simulink model "model"  (R2016a)
(part 10 of 11)

  _CN_91086220_220000_CN_24976300_220000/RConn3 -- T_24976300_380000;220000;110000_Umspannwerk_Pleinting/RConn3 -- Pleinting___Schwandorf_CN_24976300_220000_CN_28956649_220000/RConn3 -- L_24976300/LConn3
  _CN_91086220_220000_CN_77694901_220000/RConn1 -- T_77694901_220000;110000_Umspannwerk_Altheim/LConn1 -- Altheim___Sittling_CN_24759324_220000_CN_77694901_220000/LConn1
  _CN_91086220_220000_CN_77694901_220000/RConn2 -- T_77694901_220000;110000_Umspannwerk_Altheim/LConn2 -- Altheim___Sittling_CN_24759324_220000_CN_77694901_220000/LConn2
  _CN_91086220_220000_CN_77694901_220000/RConn3 -- T_77694901_220000;110000_Umspannwerk_Altheim/LConn3 -- Altheim___Sittling_CN_24759324_220000_CN_77694901_220000/LConn3
  _CN_152924498_220000_CN152506744/RConn1 -- G_152506744_Großkraftwerk_Mannheim/RConn1 -- _CN_163093653_220000_CN152506744/LConn1
  _CN_152924498_220000_CN152506744/RConn2 -- G_152506744_Großkraftwerk_Mannheim/RConn2 -- _CN_163093653_220000_CN152506744/LConn2
  _CN_152924498_220000_CN152506744/RConn3 -- G_152506744_Großkraftwerk_Mannheim/RConn3 -- _CN_163093653_220000_CN152506744/LConn3
  220kV_Fichtenhain_West+Utfort_West_CN_93278553_220000_CN_24815262_220000/LConn1 -- T_93278553_220000;110000_Station_Edelstahl_Krefeld/LConn1 -- 220kV_Fichtenhain_West+Utfort_West_CN_93278553_220000_CN_24799890_220000/RConn1 -- 220kV_Fichtenhain_West+Utfort_West_CN_93278553_220000_CN_23380800_220000/LConn1 -- 220kV_Fichtenhain_West+Utfort_West_CN_93278553_220000_CN92877616/LConn1 -- 220kV_Fichtenhain_West+Utfort_West_CN_93278553_220000_CN_91854336_220000/RConn1 -- 220kV_Fichtenhain_West+Utfort_West_CN_93278553_220000_CN_24479984_220000/LConn1
  220kV_Fichtenhain_West+Utfort_West_CN_93278553_220000_CN_24815262_220000/LConn2 -- T_93278553_220000;110000_Station_Edelstahl_Krefeld/LConn2 -- 220kV_Fichtenhain_West+Utfort_West_CN_93278553_220000_CN_24799890_220000/RConn2 -- 220kV_Fichtenhain_West+Utfort_West_CN_93278553_220000_CN_23380800_220000/LConn2 -- 220kV_Fichtenhain_West+Utfort_West_CN_93278553_220000_CN92877616/LConn2 -- 220kV_Fichtenhain_West+Utfort_West_CN_93278553_220000_CN_91854336_220000/RConn2 -- 220kV_Fichtenhain_West+Utfort_West_CN_93278553_220000_CN_24479984_220000/LConn2
  220kV_Fichtenhain_West+Utfort_West_CN_93278553_220000_CN_24815262_220000/LConn3 -- T_93278553_220000;110000_Station_Edelstahl_Krefeld/LConn3 -- 220kV_Fichtenhain_West+Utfort_West_CN_93278553_220000_CN_24799890_220000/RConn3 -- 220kV_Fichtenhain_West+Utfort_West_CN_93278553_220000_CN_23380800_220000/LConn3 -- 220kV_Fichtenhain_West+Utfort_West_CN_93278553_220000_CN92877616/LConn3 -- 220kV_Fichtenhain_West+Utfort_West_CN_93278553_220000_CN_91854336_220000/RConn3 -- 220kV_Fichtenhain_West+Utfort_West_CN_93278553_220000_CN_24479984_220000/LConn3
  220kV_Fichtenhain_West+Utfort_West_CN_93278553_220000_CN_24815262_220000/RConn1 -- T_24815262_380000;220000;110000_Station_Dülken/RConn1 -- L_24815262/LConn1
  220kV_Fichtenhain_West+Utfort_West_CN_93278553_220000_CN_24815262_220000/RConn2 -- T_24815262_380000;220000;110000_Station_Dülken/RConn2 -- L_24815262/LConn2
  220kV_Fichtenhain_West+Utfort_West_CN_93278553_220000_CN_24815262_220000/RConn3 -- T_24815262_380000;220000;110000_Station_Dülken/RConn3 -- L_24815262/LConn3
  220kV_Fichtenhain_West+Utfort_West_CN_93278553_220000_CN_23380800_220000/RConn1 -- T_23380800_380000;220000;110000_Station_Utfort/RConn1 -- 220kV_Wesel_Ost_CN_24462426_220000_CN_23380800_220000/RConn1 -- L_23380800/LConn1
  220kV_Fichtenhain_West+Utfort_West_CN_93278553_220000_CN_23380800_220000/RConn2 -- T_23380800_380000;220000;110000_Station_Utfort/RConn2 -- 220kV_Wesel_Ost_CN_24462426_220000_CN_23380800_220000/RConn2 -- L_23380800/LConn2
  220kV_Fichtenhain_West+Utfort_West_CN_93278553_220000_CN_23380800_220000/RConn3 -- T_23380800_380000;220000;110000_Station_Utfort/RConn3 -- 220kV_Wesel_Ost_CN_24462426_220000_CN_23380800_220000/RConn3 -- L_23380800/LConn3
  G_92877616_Kraftwerk_Huckingen/RConn1 -- 220kV_Fichtenhain_West+Utfort_West_CN_93278553_220000_CN92877616/RConn1
  G_92877616_Kraftwerk_Huckingen/RConn2 -- 220kV_Fichtenhain_West+Utfort_West_CN_93278553_220000_CN92877616/RConn2
  G_92877616_Kraftwerk_Huckingen/RConn3 -- 220kV_Fichtenhain_West+Utfort_West_CN_93278553_220000_CN92877616/RConn3
  T_24479984_220000;110000_Uerdingen/LConn1 -- 220kV_Fichtenhain_West+Utfort_West_CN_93278553_220000_CN_24479984_220000/RConn1
  T_24479984_220000;110000_Uerdingen/LConn2 -- 220kV_Fichtenhain_West+Utfort_West_CN_93278553_220000_CN_24479984_220000/RConn2
  T_24479984_220000;110000_Uerdingen/LConn3 -- 220kV_Fichtenhain_West+Utfort_West_CN_93278553_220000_CN_24479984_220000/RConn3
  T_74893659_380000;110000_HGÜ_Baltic_Cable___Stromrichterstation_Herrenwyk/LConn1 -- _CN_74893659_380000_CN_74893662_380000/LConn1
  T_74893659_380000;110000_HGÜ_Baltic_Cable___Stromrichterstation_Herrenwyk/LConn2 -- _CN_74893659_380000_CN_74893662_380000/LConn2
  T_74893659_380000;110000_HGÜ_Baltic_Cable___Stromrichterstation_Herrenwyk/LConn3 -- _CN_74893659_380000_CN_74893662_380000/LConn3
  T_74893662_380000;220000;110000_Umspannwerk_Siems/LConn1 -- _CN_74893659_380000_CN_74893662_380000/RConn1
  T_74893662_380000;220000;110000_Umspannwerk_Siems/LConn2 -- _CN_74893659_380000_CN_74893662_380000/RConn2
  T_74893662_380000;220000;110000_Umspannwerk_Siems/LConn3 -- _CN_74893659_380000_CN_74893662_380000/RConn3
  Scholven_C_CN_38584673_220000_CN22943608/RConn1 -- G_22943608_Kraftwerk_Scholven/RConn1 -- 220kV_Scholven_E_CN_23022100_220000_CN22943608/RConn1 -- 380kV_Scholven_B_CN_23022100_380000_CN22943608/RConn1
  Scholven_C_CN_38584673_220000_CN22943608/RConn2 -- G_22943608_Kraftwerk_Scholven/RConn2 -- 220kV_Scholven_E_CN_23022100_220000_CN22943608/RConn2 -- 380kV_Scholven_B_CN_23022100_380000_CN22943608/RConn2
  Scholven_C_CN_38584673_220000_CN22943608/RConn3 -- G_22943608_Kraftwerk_Scholven/RConn3 -- 220kV_Scholven_E_CN_23022100_220000_CN22943608/RConn3 -- 380kV_Scholven_B_CN_23022100_380000_CN22943608/RConn3
  T_89352550_380000;220000;110000_Bexbach_Kraftwerk/LConn1 -- _CN_89352550_380000_CN28051874/RConn1
  T_89352550_380000;220000;110000_Bexbach_Kraftwerk/LConn2 -- _CN_89352550_380000_CN28051874/RConn2
  T_89352550_380000;220000;110000_Bexbach_Kraftwerk/LConn3 -- _CN_89352550_380000_CN28051874/RConn3
  _CN_89352550_220000_CN28051874/RConn1 -- T_89352550_380000;220000;110000_Bexbach_Kraftwerk/RConn1 -- L_89352550/LConn1
  _CN_89352550_220000_CN28051874/RConn2 -- T_89352550_380000;220000;110000_Bexbach_Kraftwerk/RConn2 -- L_89352550/LConn2
  _CN_89352550_220000_CN28051874/RConn3 -- T_89352550_380000;220000;110000_Bexbach_Kraftwerk/RConn3 -- L_89352550/LConn3
  220_kV_Bigge_Ost|West_CN_22761839_220000_CN_24667346_220000/RConn1 -- T_24667346_220000;110000_Umspannwerk_Garenfeld/LConn1 -- _CN_66038431_220000_CN_24667346_220000/LConn1 -- 220kV_Nordleitung_CN_24667346_220000_CN_83916207_220000/LConn1
  220_kV_Bigge_Ost|West_CN_22761839_220000_CN_24667346_220000/RConn2 -- T_24667346_220000;110000_Umspannwerk_Garenfeld/LConn2 -- _CN_66038431_220000_CN_24667346_220000/LConn2 -- 220kV_Nordleitung_CN_24667346_220000_CN_83916207_220000/LConn2
  220_kV_Bigge_Ost|West_CN_22761839_220000_CN_24667346_220000/RConn3 -- T_24667346_220000;110000_Umspannwerk_Garenfeld/LConn3 -- _CN_66038431_220000_CN_24667346_220000/LConn3 -- 220kV_Nordleitung_CN_24667346_220000_CN_83916207_220000/LConn3
  T_51940126_220000;110000_Umspannwerk_Bixterheide/LConn1 -- 220_kV_Bigge_Ost|West_CN_22761839_220000_CN_51940126_220000/RConn1
  T_51940126_220000;110000_Umspannwerk_Bixterheide/LConn2 -- 220_kV_Bigge_Ost|West_CN_22761839_220000_CN_51940126_220000/RConn2
  T_51940126_220000;110000_Umspannwerk_Bixterheide/LConn3 -- 220_kV_Bigge_Ost|West_CN_22761839_220000_CN_51940126_220000/RConn3
  220_kV_Bigge_Ost|West_CN_22761839_220000_CN_132814303_220000/RConn1 -- T_132814303_220000;110000_Station_Altenkleusheim/LConn1 -- 220kV_Siegerland_West_CN_89043564_220000_CN_132814303_220000/LConn1
  220_kV_Bigge_Ost|West_CN_22761839_220000_CN_132814303_220000/RConn2 -- T_132814303_220000;110000_Station_Altenkleusheim/LConn2 -- 220kV_Siegerland_West_CN_89043564_220000_CN_132814303_220000/LConn2
  220_kV_Bigge_Ost|West_CN_22761839_220000_CN_132814303_220000/RConn3 -- T_132814303_220000;110000_Station_Altenkleusheim/LConn3 -- 220kV_Siegerland_West_CN_89043564_220000_CN_132814303_220000/LConn3
  T_22761692_220000;110000_UW_Fühlingen/LConn1 -- 220_kV_Niederaußem_4d;_Wiesdorf_Ltg__CN_22761839_220000_CN_22761692_220000/RConn1
  T_22761692_220000;110000_UW_Fühlingen/LConn2 -- 220_kV_Niederaußem_4d;_Wiesdorf_Ltg__CN_22761839_220000_CN_22761692_220000/RConn2
  T_22761692_220000;110000_UW_Fühlingen/LConn3 -- 220_kV_Niederaußem_4d;_Wiesdorf_Ltg__CN_22761839_220000_CN_22761692_220000/RConn3
  220_kV_Niederaußem_4d;_Wiesdorf_Ltg__CN_22761839_220000_CN_24839976_220000/RConn1 -- T_24839976_380000;220000_Umspannwerk_Rommerskirchen/RConn1 -- 220_kV_Rommerskirchen_Ost_CN_24839976_220000_CN_23084554_220000/LConn1 -- 220_kV_Frixheim_Nord|Süd_CN_24839976_220000_CN_27919734_220000/LConn1 -- L_24839976/LConn1
  220_kV_Niederaußem_4d;_Wiesdorf_Ltg__CN_22761839_220000_CN_24839976_220000/RConn2 -- T_24839976_380000;220000_Umspannwerk_Rommerskirchen/RConn2 -- 220_kV_Rommerskirchen_Ost_CN_24839976_220000_CN_23084554_220000/LConn2 -- 220_kV_Frixheim_Nord|Süd_CN_24839976_220000_CN_27919734_220000/LConn2 -- L_24839976/LConn2
  220_kV_Niederaußem_4d;_Wiesdorf_Ltg__CN_22761839_220000_CN_24839976_220000/RConn3 -- T_24839976_380000;220000_Umspannwerk_Rommerskirchen/RConn3 -- 220_kV_Rommerskirchen_Ost_CN_24839976_220000_CN_23084554_220000/LConn3 -- 220_kV_Frixheim_Nord|Süd_CN_24839976_220000_CN_27919734_220000/LConn3 -- L_24839976/LConn3
  220_kV_Niederaußem_4d;_Wiesdorf_Ltg__CN_22761839_220000_CN24840439/RConn1 -- G_24840439_Kraftwerk_Niederaussem/RConn1 -- 220_kV_Niederaußem_3c_CN_32993727_220000_CN24840439/LConn1 -- _CN_24839976_380000_CN24840439/RConn1
  220_kV_Niederaußem_4d;_Wiesdorf_Ltg__CN_22761839_220000_CN24840439/RConn2 -- G_24840439_Kraftwerk_Niederaussem/RConn2 -- 220_kV_Niederaußem_3c_CN_32993727_220000_CN24840439/LConn2 -- _CN_24839976_380000_CN24840439/RConn2
  220_kV_Niederaußem_4d;_Wiesdorf_Ltg__CN_22761839_220000_CN24840439/RConn3 -- G_24840439_Kraftwerk_Niederaussem/RConn3 -- 220_kV_Niederaußem_3c_CN_32993727_220000_CN24840439/LConn3 -- _CN_24839976_380000_CN24840439/RConn3
  T_22764922_220000;110000_Station_Dhünnaue/LConn1 -- 220_kV_Niederaußem_4d;_Wiesdorf_Ltg__CN_22761839_220000_CN_22764922_220000/RConn1
  T_22764922_220000;110000_Station_Dhünnaue/LConn2 -- 220_kV_Niederaußem_4d;_Wiesdorf_Ltg__CN_22761839_220000_CN_22764922_220000/RConn2
  T_22764922_220000;110000_Station_Dhünnaue/LConn3 -- 220_kV_Niederaußem_4d;_Wiesdorf_Ltg__CN_22761839_220000_CN_22764922_220000/RConn3
  380_kV_Neurath_2b;_Oerkhaus_Ost_CN_22761839_380000_CN_49577448_380000/RConn1 -- T_49577448_380000;220000_Station_Sankt_Peter_380_kV/LConn1 -- 380kV_Knechtsteden_West_CN_77179271_380000_CN_49577448_380000/LConn1
  380_kV_Neurath_2b;_Oerkhaus_Ost_CN_22761839_380000_CN_49577448_380000/RConn2 -- T_49577448_380000;220000_Station_Sankt_Peter_380_kV/LConn2 -- 380kV_Knechtsteden_West_CN_77179271_380000_CN_49577448_380000/LConn2
  380_kV_Neurath_2b;_Oerkhaus_Ost_CN_22761839_380000_CN_49577448_380000/RConn3 -- T_49577448_380000;220000_Station_Sankt_Peter_380_kV/LConn3 -- 380kV_Knechtsteden_West_CN_77179271_380000_CN_49577448_380000/LConn3
  T_106096507_380000;110000_Station_Ohligs/LConn1 -- 380_kV_Neurath_2b;_Oerkhaus_Ost_CN_22761839_380000_CN_106096507_380000/RConn1
  T_106096507_380000;110000_Station_Ohligs/LConn2 -- 380_kV_Neurath_2b;_Oerkhaus_Ost_CN_22761839_380000_CN_106096507_380000/RConn2
  T_106096507_380000;110000_Station_Ohligs/LConn3 -- 380_kV_Neurath_2b;_Oerkhaus_Ost_CN_22761839_380000_CN_106096507_380000/RConn3
  380kV_Sauerland_Süd_CN_42799487_380000_CN_42488850_380000/RConn1 -- T_42799487_380000;110000_Station_Arpe/LConn1 -- 380kV_Sauerland_Süd_CN_42799487_380000_CN_42797575_380000/LConn1
  380kV_Sauerland_Süd_CN_42799487_380000_CN_42488850_380000/RConn2 -- T_42799487_380000;110000_Station_Arpe/LConn2 -- 380kV_Sauerland_Süd_CN_42799487_380000_CN_42797575_380000/LConn2
  380kV_Sauerland_Süd_CN_42799487_380000_CN_42488850_380000/RConn3 -- T_42799487_380000;110000_Station_Arpe/LConn3 -- 380kV_Sauerland_Süd_CN_42799487_380000_CN_42797575_380000/LConn3
  380kV_Sauerland_Süd_CN_42799487_380000_CN_42797575_380000/RConn1 -- T_42797575_380000;110000_Station_Nehden/LConn1 -- 380kV_Twistetal_Ost_3_CN_42797575_380000_CN_41232144_380000/LConn1 -- 380kV_Twistetal_Ost_3_CN_42797575_380000_CN_25943440_380000/LConn1
  380kV_Sauerland_Süd_CN_42799487_380000_CN_42797575_380000/RConn2 -- T_42797575_380000;110000_Station_Nehden/LConn2 -- 380kV_Twistetal_Ost_3_CN_42797575_380000_CN_41232144_380000/LConn2 -- 380kV_Twistetal_Ost_3_CN_42797575_380000_CN_25943440_380000/LConn2
  380kV_Sauerland_Süd_CN_42799487_380000_CN_42797575_380000/RConn3 -- T_42797575_380000;110000_Station_Nehden/LConn3 -- 380kV_Twistetal_Ost_3_CN_42797575_380000_CN_41232144_380000/LConn3 -- 380kV_Twistetal_Ost_3_CN_42797575_380000_CN_25943440_380000/LConn3
  380kV_Knechtsteden_West_CN_77179271_380000_CN_24839976_380000/RConn1 -- T_77179271_380000_Station_Osterath/LConn1 -- 380kV_Meerbusch_West_CN_77179271_380000_CN_25044557_380000/LConn1 -- 380kV_Knechtsteden_West_CN_77179271_380000_CN_49577448_380000/RConn1 -- 380kV_Knechtsteden_West_CN_77179271_380000_CN_95434457_380000/LConn1 -- 380kV_Knechtsteden_West_CN_77179271_380000_CN109373271/LConn1 -- 380kV_Meerbusch_West_CN_77179271_380000_CN_23380800_380000/LConn1
  380kV_Knechtsteden_West_CN_77179271_380000_CN_24839976_380000/RConn2 -- T_77179271_380000_Station_Osterath/LConn2 -- 380kV_Meerbusch_West_CN_77179271_380000_CN_25044557_380000/LConn2 -- 380kV_Knechtsteden_West_CN_77179271_380000_CN_49577448_380000/RConn2 -- 380kV_Knechtsteden_West_CN_77179271_380000_CN_95434457_380000/LConn2 -- 380kV_Knechtsteden_West_CN_77179271_380000_CN109373271/LConn2 -- 380kV_Meerbusch_West_CN_77179271_380000_CN_23380800_380000/LConn2
  380kV_Knechtsteden_West_CN_77179271_380000_CN_24839976_380000/RConn3 -- T_77179271_380000_Station_Osterath/LConn3 -- 380kV_Meerbusch_West_CN_77179271_380000_CN_25044557_380000/LConn3 -- 380kV_Knechtsteden_West_CN_77179271_380000_CN_49577448_380000/RConn3 -- 380kV_Knechtsteden_West_CN_77179271_380000_CN_95434457_380000/LConn3 -- 380kV_Knechtsteden_West_CN_77179271_380000_CN109373271/LConn3 -- 380kV_Meerbusch_West_CN_77179271_380000_CN_23380800_380000/LConn3
  T_95434457_380000;220000;110000_KW_Neurath/LConn1 -- 380kV_Knechtsteden_West_CN_77179271_380000_CN_95434457_380000/RConn1
  T_95434457_380000;220000;110000_KW_Neurath/LConn2 -- 380kV_Knechtsteden_West_CN_77179271_380000_CN_95434457_380000/RConn2
  T_95434457_380000;220000;110000_KW_Neurath/LConn3 -- 380kV_Knechtsteden_West_CN_77179271_380000_CN_95434457_380000/RConn3
  G_109373271_RWE_Kraftwerk_Neurath_BoA_Bl__F_G/RConn1 -- 380kV_Knechtsteden_West_CN_77179271_380000_CN109373271/RConn1
  G_109373271_RWE_Kraftwerk_Neurath_BoA_Bl__F_G/RConn2 -- 380kV_Knechtsteden_West_CN_77179271_380000_CN109373271/RConn2
  G_109373271_RWE_Kraftwerk_Neurath_BoA_Bl__F_G/RConn3 -- 380kV_Knechtsteden_West_CN_77179271_380000_CN109373271/RConn3
  380kV_Meerbusch_West_CN_77179271_380000_CN_23380800_380000/RConn1 -- T_23380800_380000;220000;110000_Station_Utfort/LConn1 -- 380kV_Lohheide_West_CN_23380800_380000_CN26623135/RConn1
  380kV_Meerbusch_West_CN_77179271_380000_CN_23380800_380000/RConn2 -- T_23380800_380000;220000;110000_Station_Utfort/LConn2 -- 380kV_Lohheide_West_CN_23380800_380000_CN26623135/RConn2
  380kV_Meerbusch_West_CN_77179271_380000_CN_23380800_380000/RConn3 -- T_23380800_380000;220000;110000_Station_Utfort/LConn3 -- 380kV_Lohheide_West_CN_23380800_380000_CN26623135/RConn3
  T_25044557_380000_Station_Rath/LConn1 -- 380kV_Meerbusch_West_CN_77179271_380000_CN_25044557_380000/RConn1
  T_25044557_380000_Station_Rath/LConn2 -- 380kV_Meerbusch_West_CN_77179271_380000_CN_25044557_380000/RConn2
  T_25044557_380000_Station_Rath/LConn3 -- 380kV_Meerbusch_West_CN_77179271_380000_CN_25044557_380000/RConn3
  G_178167136_Kraftwerk_Boxberg/RConn1 -- MP_CN_157806991_380000_CN178167136/RConn1
  G_178167136_Kraftwerk_Boxberg/RConn2 -- MP_CN_157806991_380000_CN178167136/RConn2
  G_178167136_Kraftwerk_Boxberg/RConn3 -- MP_CN_157806991_380000_CN178167136/RConn3
  557_CN_157806991_380000_CN_157328339_380000/RConn1 -- T_157328339_380000;110000_Umspannwerk_Streumen/LConn1 -- 585_CN_157328339_380000_CN_32843531_380000/RConn1 -- 559_CN_157328339_380000_CN_23025610_380000/RConn1 -- 572_CN_23117075_380000_CN_157328339_380000/RConn1 -- 561_Streumen_CN_156683994_380000_CN_157328339_380000/RConn1
  557_CN_157806991_380000_CN_157328339_380000/RConn2 -- T_157328339_380000;110000_Umspannwerk_Streumen/LConn2 -- 585_CN_157328339_380000_CN_32843531_380000/RConn2 -- 559_CN_157328339_380000_CN_23025610_380000/RConn2 -- 572_CN_23117075_380000_CN_157328339_380000/RConn2 -- 561_Streumen_CN_156683994_380000_CN_157328339_380000/RConn2
  557_CN_157806991_380000_CN_157328339_380000/RConn3 -- T_157328339_380000;110000_Umspannwerk_Streumen/LConn3 -- 585_CN_157328339_380000_CN_32843531_380000/RConn3 -- 559_CN_157328339_380000_CN_23025610_380000/RConn3 -- 572_CN_23117075_380000_CN_157328339_380000/RConn3 -- 561_Streumen_CN_156683994_380000_CN_157328339_380000/RConn3
  552_CN_157806991_380000_CN_157807291_380000/RConn1 -- T_157807291_380000;110000_Umspannwerk_Schmölln/LConn1 -- Schmölln___Dresden_Süd___Röhrsdorf_CN_157807291_380000_CN_109917397_380000/LConn1 -- Schmölln___Dresden_Süd___Röhrsdorf_CN_157807291_380000_CN_23117075_380000/RConn1 -- Schmölln___Dresden_Süd___Röhrsdorf_CN_157807291_380000_CN_23241863_380000/LConn1 -- _CN_59026005_380000_CN_157807291_380000/LConn1
  552_CN_157806991_380000_CN_157807291_380000/RConn2 -- T_157807291_380000;110000_Umspannwerk_Schmölln/LConn2 -- Schmölln___Dresden_Süd___Röhrsdorf_CN_157807291_380000_CN_109917397_380000/LConn2 -- Schmölln___Dresden_Süd___Röhrsdorf_CN_157807291_380000_CN_23117075_380000/RConn2 -- Schmölln___Dresden_Süd___Röhrsdorf_CN_157807291_380000_CN_23241863_380000/LConn2 -- _CN_59026005_380000_CN_157807291_380000/LConn2
  552_CN_157806991_380000_CN_157807291_380000/RConn3 -- T_157807291_380000;110000_Umspannwerk_Schmölln/LConn3 -- Schmölln___Dresden_Süd___Röhrsdorf_CN_157807291_380000_CN_109917397_380000/LConn3 -- Schmölln___Dresden_Süd___Röhrsdorf_CN_157807291_380000_CN_23117075_380000/RConn3 -- Schmölln___Dresden_Süd___Röhrsdorf_CN_157807291_380000_CN_23241863_380000/LConn3 -- _CN_59026005_380000_CN_157807291_380000/LConn3
  _CN_25557397_380000_CN_43688805_380000/RConn1 -- T_43688805_380000;220000;110000_380kV_Umspannwerk_Pulverdingen/LConn1 -- Philippsburg___Pulverdingen_CN_43688805_380000_CN_254326606_380000/LConn1 -- Philippsburg___Pulverdingen_CN_43688805_380000_CN161909939/RConn1 -- 380_kV_CN_26260052_380000_CN_43688805_380000/LConn1 -- 2x_380_kV_CN_43688805_380000_CN_26814283_380000/LConn1
  _CN_25557397_380000_CN_43688805_380000/RConn2 -- T_43688805_380000;220000;110000_380kV_Umspannwerk_Pulverdingen/LConn2 -- Philippsburg___Pulverdingen_CN_43688805_380000_CN_254326606_380000/LConn2 -- Philippsburg___Pulverdingen_CN_43688805_380000_CN161909939/RConn2 -- 380_kV_CN_26260052_380000_CN_43688805_380000/LConn2 -- 2x_380_kV_CN_43688805_380000_CN_26814283_380000/LConn2
  _CN_25557397_380000_CN_43688805_380000/RConn3 -- T_43688805_380000;220000;110000_380kV_Umspannwerk_Pulverdingen/LConn3 -- Philippsburg___Pulverdingen_CN_43688805_380000_CN_254326606_380000/LConn3 -- Philippsburg___Pulverdingen_CN_43688805_380000_CN161909939/RConn3 -- 380_kV_CN_26260052_380000_CN_43688805_380000/LConn3 -- 2x_380_kV_CN_43688805_380000_CN_26814283_380000/LConn3
  G_146723308_Kernkraftwerk_Obrigheim,_stillgelegt/RConn1 -- _CN_25557397_220000_CN146723308/RConn1
  G_146723308_Kernkraftwerk_Obrigheim,_stillgelegt/RConn2 -- _CN_25557397_220000_CN146723308/RConn2
  G_146723308_Kernkraftwerk_Obrigheim,_stillgelegt/RConn3 -- _CN_25557397_220000_CN146723308/RConn3
  _CN_25557397_220000_CN_42050342_220000/RConn1 -- T_42050342_380000;220000;110000_Umspannwerk_Goldshöfe/RConn1 -- L_42050342/LConn1
  _CN_25557397_220000_CN_42050342_220000/RConn2 -- T_42050342_380000;220000;110000_Umspannwerk_Goldshöfe/RConn2 -- L_42050342/LConn2
  _CN_25557397_220000_CN_42050342_220000/RConn3 -- T_42050342_380000;220000;110000_Umspannwerk_Goldshöfe/RConn3 -- L_42050342/LConn3
  _CN_25557397_380000_CN89183108/RConn1 -- G_89183108_Heizkraftwerk_Heilbronn/RConn1 -- _CN_25557397_220000_CN89183108/RConn1
  _CN_25557397_380000_CN89183108/RConn2 -- G_89183108_Heizkraftwerk_Heilbronn/RConn2 -- _CN_25557397_220000_CN89183108/RConn2
  _CN_25557397_380000_CN89183108/RConn3 -- G_89183108_Heizkraftwerk_Heilbronn/RConn3 -- _CN_25557397_220000_CN89183108/RConn3
  T_104878489_220000;110000_Umspannwerk_Kraftwerk_Emden/LConn1 -- _CN_104878489_220000_CN_34835258_220000/LConn1
  T_104878489_220000;110000_Umspannwerk_Kraftwerk_Emden/LConn2 -- _CN_104878489_220000_CN_34835258_220000/LConn2
  T_104878489_220000;110000_Umspannwerk_Kraftwerk_Emden/LConn3 -- _CN_104878489_220000_CN_34835258_220000/LConn3
  _CN_104878489_220000_CN_34835258_220000/RConn1 -- T_34835258_220000;110000_Emden_Borßum/LConn1 -- 203_CN_34835258_220000_CN_173178563_220000/LConn1
  _CN_104878489_220000_CN_34835258_220000/RConn2 -- T_34835258_220000;110000_Emden_Borßum/LConn2 -- 203_CN_34835258_220000_CN_173178563_220000/LConn2
  _CN_104878489_220000_CN_34835258_220000/RConn3 -- T_34835258_220000;110000_Emden_Borßum/LConn3 -- 203_CN_34835258_220000_CN_173178563_220000/LConn3
  Wolkramshausen_CN_143882655_220000_CN_157164284_220000/LConn1 -- T_143882655_380000;220000;110000_Umspannwerk_Vieselbach/RConn1 -- L_143882655/LConn1
  Wolkramshausen_CN_143882655_220000_CN_157164284_220000/LConn2 -- T_143882655_380000;220000;110000_Umspannwerk_Vieselbach/RConn2 -- L_143882655/LConn2
  Wolkramshausen_CN_143882655_220000_CN_157164284_220000/LConn3 -- T_143882655_380000;220000;110000_Umspannwerk_Vieselbach/RConn3 -- L_143882655/LConn3
  Wolkramshausen_CN_143882655_220000_CN_157164284_220000/RConn1 -- T_157164284_220000_Wolkramshausen_(220_kV)/LConn1 -- 358_CN_157164284_220000_CN_22879599_220000/LConn1
  Wolkramshausen_CN_143882655_220000_CN_157164284_220000/RConn2 -- T_157164284_220000_Wolkramshausen_(220_kV)/LConn2 -- 358_CN_157164284_220000_CN_22879599_220000/LConn2
  Wolkramshausen_CN_143882655_220000_CN_157164284_220000/RConn3 -- T_157164284_220000_Wolkramshausen_(220_kV)/LConn3 -- 358_CN_157164284_220000_CN_22879599_220000/LConn3
  _CN_143882655_380000_CN_29309786_380000/RConn1 -- T_29309786_380000;110000_Mecklar/LConn1 -- _CN_29309786_380000_CN_156673636_380000/LConn1 -- _CN_29309786_380000_CN_148446247_380000/LConn1
  _CN_143882655_380000_CN_29309786_380000/RConn2 -- T_29309786_380000;110000_Mecklar/LConn2 -- _CN_29309786_380000_CN_156673636_380000/LConn2 -- _CN_29309786_380000_CN_148446247_380000/LConn2
  _CN_143882655_380000_CN_29309786_380000/RConn3 -- T_29309786_380000;110000_Mecklar/LConn3 -- _CN_29309786_380000_CN_156673636_380000/LConn3 -- _CN_29309786_380000_CN_148446247_380000/LConn3
  T_154418450_380000;110000_Eisenach/LConn1 -- _CN_143882655_380000_CN_154418450_380000/RConn1
  T_154418450_380000;110000_Eisenach/LConn2 -- _CN_143882655_380000_CN_154418450_380000/RConn2
  T_154418450_380000;110000_Eisenach/LConn3 -- _CN_143882655_380000_CN_154418450_380000/RConn3
  T_148211527_380000;110000_Großschwabhausen/LConn1 -- _CN_143882655_380000_CN_148211527_380000/RConn1
  T_148211527_380000;110000_Großschwabhausen/LConn2 -- _CN_143882655_380000_CN_148211527_380000/RConn2
  T_148211527_380000;110000_Großschwabhausen/LConn3 -- _CN_143882655_380000_CN_148211527_380000/RConn3
  T_24267175_220000;110000_Umspannanlage_Frimmersdorf_I/LConn1 -- _CN_24267175_220000_CN24267119/LConn1
  T_24267175_220000;110000_Umspannanlage_Frimmersdorf_I/LConn2 -- _CN_24267175_220000_CN24267119/LConn2
  T_24267175_220000;110000_Umspannanlage_Frimmersdorf_I/LConn3 -- _CN_24267175_220000_CN24267119/LConn3
  _CN_24267175_220000_CN24267119/RConn1 -- G_24267119_RWE_Kraftwerk_Frimmersdorf/RConn1 -- 220_kV_Neurath_1a_CN_27919734_220000_CN24267119/LConn1
  _CN_24267175_220000_CN24267119/RConn2 -- G_24267119_RWE_Kraftwerk_Frimmersdorf/RConn2 -- 220_kV_Neurath_1a_CN_27919734_220000_CN24267119/LConn2
  _CN_24267175_220000_CN24267119/RConn3 -- G_24267119_RWE_Kraftwerk_Frimmersdorf/RConn3 -- 220_kV_Neurath_1a_CN_27919734_220000_CN24267119/LConn3
  T_151507370_220000_/LConn1 -- _CN_151507370_220000_CN_28227099_220000/RConn1
  T_151507370_220000_/LConn2 -- _CN_151507370_220000_CN_28227099_220000/RConn2
  T_151507370_220000_/LConn3 -- _CN_151507370_220000_CN_28227099_220000/RConn3
  T_266684854_380000_Umspannwerk_Farge/LConn1 -- _CN_266684854_380000_CN313937042/RConn1
  T_266684854_380000_Umspannwerk_Farge/LConn2 -- _CN_266684854_380000_CN313937042/RConn2
  T_266684854_380000_Umspannwerk_Farge/LConn3 -- _CN_266684854_380000_CN313937042/RConn3
  _CN_68532663_220000_CN252655527/LConn1 -- T_68532663_220000;110000_Umspannwerk_Krün/LConn1 -- _CN_68532663_220000_CN_24237879_220000/LConn1
  _CN_68532663_220000_CN252655527/LConn2 -- T_68532663_220000;110000_Umspannwerk_Krün/LConn2 -- _CN_68532663_220000_CN_24237879_220000/LConn2
  _CN_68532663_220000_CN252655527/LConn3 -- T_68532663_220000;110000_Umspannwerk_Krün/LConn3 -- _CN_68532663_220000_CN_24237879_220000/LConn3
  G_252655527_Stauwehr_Krün/RConn1 -- _CN_68532663_220000_CN252655527/RConn1
  G_252655527_Stauwehr_Krün/RConn2 -- _CN_68532663_220000_CN252655527/RConn2
  G_252655527_Stauwehr_Krün/RConn3 -- _CN_68532663_220000_CN252655527/RConn3
  _CN_68532663_220000_CN_24237879_220000/RConn1 -- T_24237879_220000;110000_Umspannwerk_Oberbrunn/LConn1 -- Oberbrunn___Oberbachern_CN_18629425_220000_CN_24237879_220000/RConn1
  _CN_68532663_220000_CN_24237879_220000/RConn2 -- T_24237879_220000;110000_Umspannwerk_Oberbrunn/LConn2 -- Oberbrunn___Oberbachern_CN_18629425_220000_CN_24237879_220000/RConn2
  _CN_68532663_220000_CN_24237879_220000/RConn3 -- T_24237879_220000;110000_Umspannwerk_Oberbrunn/LConn3 -- Oberbrunn___Oberbachern_CN_18629425_220000_CN_24237879_220000/RConn3
  T_32993727_220000;110000_KW_Niederaußem/LConn1 -- 220_kV_Niederaußem_3c_CN_32993727_220000_CN24840439/RConn1
  T_32993727_220000;110000_KW_Niederaußem/LConn2 -- 220_kV_Niederaußem_3c_CN_32993727_220000_CN24840439/RConn2
  T_32993727_220000;110000_KW_Niederaußem/LConn3 -- 220_kV_Niederaußem_3c_CN_32993727_220000_CN24840439/RConn3
  _CN_35833592_220000_CN_35833442_220000/RConn1 -- T_35833442_220000_/LConn1 -- _CN_35833442_220000_CN125808869/LConn1
  _CN_35833592_220000_CN_35833442_220000/RConn2 -- T_35833442_220000_/LConn2 -- _CN_35833442_220000_CN125808869/LConn2
  _CN_35833592_220000_CN_35833442_220000/RConn3 -- T_35833442_220000_/LConn3 -- _CN_35833442_220000_CN125808869/LConn3
  T_158253525_220000;110000_Umspannwerk_Paderborn_Süd/LConn1 -- _CN_158253525_220000_CN_24264701_220000/RConn1
  T_158253525_220000;110000_Umspannwerk_Paderborn_Süd/LConn2 -- _CN_158253525_220000_CN_24264701_220000/RConn2
  T_158253525_220000;110000_Umspannwerk_Paderborn_Süd/LConn3 -- _CN_158253525_220000_CN_24264701_220000/RConn3
  493_CN_26472665_380000_CN_30132758_380000/RConn1 -- T_30132758_380000;110000_Teufelsbruch/LConn1 -- _CN_30132758_380000_CN_43163132_380000/LConn1
  493_CN_26472665_380000_CN_30132758_380000/RConn2 -- T_30132758_380000;110000_Teufelsbruch/LConn2 -- _CN_30132758_380000_CN_43163132_380000/LConn2
  493_CN_26472665_380000_CN_30132758_380000/RConn3 -- T_30132758_380000;110000_Teufelsbruch/LConn3 -- _CN_30132758_380000_CN_43163132_380000/LConn3
  T_32690742_380000;110000_Umspannwerk_Klostermansfeld/LConn1 -- 536_CN_26472665_380000_CN_32690742_380000/RConn1
  T_32690742_380000;110000_Umspannwerk_Klostermansfeld/LConn2 -- 536_CN_26472665_380000_CN_32690742_380000/RConn2
  T_32690742_380000;110000_Umspannwerk_Klostermansfeld/LConn3 -- 536_CN_26472665_380000_CN_32690742_380000/RConn3
  _CN_24414688_220000_CN_42507488_220000/RConn1 -- T_24414688_220000;110000_Station_Wambel/LConn1 -- _CN_24414688_220000_CN_24858617_220000/LConn1
  _CN_24414688_220000_CN_42507488_220000/RConn2 -- T_24414688_220000;110000_Station_Wambel/LConn2 -- _CN_24414688_220000_CN_24858617_220000/LConn2
  _CN_24414688_220000_CN_42507488_220000/RConn3 -- T_24414688_220000;110000_Station_Wambel/LConn3 -- _CN_24414688_220000_CN_24858617_220000/LConn3
  T_24858617_220000_Ratsbusch/LConn1 -- _CN_24414688_220000_CN_24858617_220000/RConn1
  T_24858617_220000_Ratsbusch/LConn2 -- _CN_24414688_220000_CN_24858617_220000/RConn2
  T_24858617_220000_Ratsbusch/LConn3 -- _CN_24414688_220000_CN_24858617_220000/RConn3
  Meitingen_Nord;_Süd_CN_24652261_380000_CN_88945213_380000/RConn1 -- T_88945213_380000_Umspannwerk_Gundelfingen/LConn1 -- _CN_88945213_380000_CN31023006/LConn1 -- _CN_88945213_380000_CN_31019939_380000/LConn1
  Meitingen_Nord;_Süd_CN_24652261_380000_CN_88945213_380000/RConn2 -- T_88945213_380000_Umspannwerk_Gundelfingen/LConn2 -- _CN_88945213_380000_CN31023006/LConn2 -- _CN_88945213_380000_CN_31019939_380000/LConn2
  Meitingen_Nord;_Süd_CN_24652261_380000_CN_88945213_380000/RConn3 -- T_88945213_380000_Umspannwerk_Gundelfingen/LConn3 -- _CN_88945213_380000_CN31023006/LConn3 -- _CN_88945213_380000_CN_31019939_380000/LConn3
  T_76246159_380000;110000_Umspannwerk_Meitingen/LConn1 -- _CN_24652261_380000_CN_76246159_380000/RConn1
  T_76246159_380000;110000_Umspannwerk_Meitingen/LConn2 -- _CN_24652261_380000_CN_76246159_380000/RConn2
  T_76246159_380000;110000_Umspannwerk_Meitingen/LConn3 -- _CN_24652261_380000_CN_76246159_380000/RConn3
  358_CN_157164284_220000_CN_22879599_220000/RConn1 -- T_22879599_220000;110000_Umspannwerk_Großdalzig/LConn1 -- _CN_22879599_220000_CN_32843531_220000/LConn1
  358_CN_157164284_220000_CN_22879599_220000/RConn2 -- T_22879599_220000;110000_Umspannwerk_Großdalzig/LConn2 -- _CN_22879599_220000_CN_32843531_220000/LConn2
  358_CN_157164284_220000_CN_22879599_220000/RConn3 -- T_22879599_220000;110000_Umspannwerk_Großdalzig/LConn3 -- _CN_22879599_220000_CN_32843531_220000/LConn3
  T_229500139_220000_DOW/LConn1 -- _CN_151765495_220000_CN_229500139_220000/RConn1
  T_229500139_220000_DOW/LConn2 -- _CN_151765495_220000_CN_229500139_220000/RConn2
  T_229500139_220000_DOW/LConn3 -- _CN_151765495_220000_CN_229500139_220000/RConn3
  419_Krümmel___Görries_CN_30040568_380000_CN_23366603_380000/LConn1 -- T_30040568_380000;110000_Görries/LConn1 -- 419_Krümmel___Görries_CN_30040568_380000_CN_234171369_380000/LConn1 -- 419_Krümmel___Görries_CN_30040568_380000_CN_32062544_380000/RConn1
  419_Krümmel___Görries_CN_30040568_380000_CN_23366603_380000/LConn2 -- T_30040568_380000;110000_Görries/LConn2 -- 419_Krümmel___Görries_CN_30040568_380000_CN_234171369_380000/LConn2 -- 419_Krümmel___Görries_CN_30040568_380000_CN_32062544_380000/RConn2
  419_Krümmel___Görries_CN_30040568_380000_CN_23366603_380000/LConn3 -- T_30040568_380000;110000_Görries/LConn3 -- 419_Krümmel___Görries_CN_30040568_380000_CN_234171369_380000/LConn3 -- 419_Krümmel___Görries_CN_30040568_380000_CN_32062544_380000/RConn3
  419_Krümmel___Görries_CN_30040568_380000_CN_23366603_380000/RConn1 -- T_23366603_380000;110000_Krümmel/LConn1 -- KKW_Krümmel___UW_HH_OST_CN_23366603_380000_CN_23583867_380000/RConn1 -- _CN_23366603_380000_CN_28327356_380000/LConn1
  419_Krümmel___Görries_CN_30040568_380000_CN_23366603_380000/RConn2 -- T_23366603_380000;110000_Krümmel/LConn2 -- KKW_Krümmel___UW_HH_OST_CN_23366603_380000_CN_23583867_380000/RConn2 -- _CN_23366603_380000_CN_28327356_380000/LConn2
  419_Krümmel___Görries_CN_30040568_380000_CN_23366603_380000/RConn3 -- T_23366603_380000;110000_Krümmel/LConn3 -- KKW_Krümmel___UW_HH_OST_CN_23366603_380000_CN_23583867_380000/RConn3 -- _CN_23366603_380000_CN_28327356_380000/LConn3
  T_234171369_380000_Wessin/LConn1 -- 419_Krümmel___Görries_CN_30040568_380000_CN_234171369_380000/RConn1
  T_234171369_380000_Wessin/LConn2 -- 419_Krümmel___Görries_CN_30040568_380000_CN_234171369_380000/RConn2
  T_234171369_380000_Wessin/LConn3 -- 419_Krümmel___Görries_CN_30040568_380000_CN_234171369_380000/RConn3
  380kV_Twistetal_Ost_3_CN_42797575_380000_CN_41232144_380000/RConn1 -- T_41232144_380000;110000_Umspannwerk_Twistetal/LConn1 -- Leitung_3212;Leitung_3213_CN_156673636_380000_CN_41232144_380000/LConn1
  380kV_Twistetal_Ost_3_CN_42797575_380000_CN_41232144_380000/RConn2 -- T_41232144_380000;110000_Umspannwerk_Twistetal/LConn2 -- Leitung_3212;Leitung_3213_CN_156673636_380000_CN_41232144_380000/LConn2
  380kV_Twistetal_Ost_3_CN_42797575_380000_CN_41232144_380000/RConn3 -- T_41232144_380000;110000_Umspannwerk_Twistetal/LConn3 -- Leitung_3212;Leitung_3213_CN_156673636_380000_CN_41232144_380000/LConn3
  380kV_Twistetal_Ost_3_CN_42797575_380000_CN_25943440_380000/RConn1 -- T_25943440_380000;110000_Umspannwerk_Elsen/LConn1 -- _CN_25943440_380000_CN_24264701_380000/LConn1
  380kV_Twistetal_Ost_3_CN_42797575_380000_CN_25943440_380000/RConn2 -- T_25943440_380000;110000_Umspannwerk_Elsen/LConn2 -- _CN_25943440_380000_CN_24264701_380000/LConn2
  380kV_Twistetal_Ost_3_CN_42797575_380000_CN_25943440_380000/RConn3 -- T_25943440_380000;110000_Umspannwerk_Elsen/LConn3 -- _CN_25943440_380000_CN_24264701_380000/LConn3
  _CN_152261133_220000_CN_163093653_220000/RConn1 -- T_163093653_220000;110000_Mannheim/LConn1 -- _CN_163093653_220000_CN152506744/RConn1
  _CN_152261133_220000_CN_163093653_220000/RConn2 -- T_163093653_220000;110000_Mannheim/LConn2 -- _CN_163093653_220000_CN152506744/RConn2
  _CN_152261133_220000_CN_163093653_220000/RConn3 -- T_163093653_220000;110000_Mannheim/LConn3 -- _CN_163093653_220000_CN152506744/RConn3
  T_160929097_220000;110000_Umspannwerk_Weinheim/LConn1 -- _CN_152261133_220000_CN_160929097_220000/RConn1
  T_160929097_220000;110000_Umspannwerk_Weinheim/LConn2 -- _CN_152261133_220000_CN_160929097_220000/RConn2
  T_160929097_220000;110000_Umspannwerk_Weinheim/LConn3 -- _CN_152261133_220000_CN_160929097_220000/RConn3
  T_154729020_220000;110000_Umspannwerk_Altlußheim/LConn1 -- _CN_152261133_220000_CN_154729020_220000/RConn1
  T_154729020_220000;110000_Umspannwerk_Altlußheim/LConn2 -- _CN_152261133_220000_CN_154729020_220000/RConn2
  T_154729020_220000;110000_Umspannwerk_Altlußheim/LConn3 -- _CN_152261133_220000_CN_154729020_220000/RConn3
  _CN_152261133_380000_CN_149987048_380000/RConn1 -- T_149987048_380000;220000_Station_Bürstadt/LConn1 -- 2_x_380_kV;_3_x_220_kV_CN_23284340_380000_CN_149987048_380000/LConn1 -- _CN_160584794_380000_CN_149987048_380000/LConn1 -- _CN_25802269_380000_CN_149987048_380000/LConn1
  _CN_152261133_380000_CN_149987048_380000/RConn2 -- T_149987048_380000;220000_Station_Bürstadt/LConn2 -- 2_x_380_kV;_3_x_220_kV_CN_23284340_380000_CN_149987048_380000/LConn2 -- _CN_160584794_380000_CN_149987048_380000/LConn2 -- _CN_25802269_380000_CN_149987048_380000/LConn2
  _CN_152261133_380000_CN_149987048_380000/RConn3 -- T_149987048_380000;220000_Station_Bürstadt/LConn3 -- 2_x_380_kV;_3_x_220_kV_CN_23284340_380000_CN_149987048_380000/LConn3 -- _CN_160584794_380000_CN_149987048_380000/LConn3 -- _CN_25802269_380000_CN_149987048_380000/LConn3
  _CN_152261133_380000_CN_54359256_380000/RConn1 -- T_54359256_380000;220000;110000_Umspannwerk_Uchtelfangen/LConn1 -- _CN_54359256_380000_CN115145869/LConn1 -- 380_kV_Gilzem_Ost;_Uchtelfangen_Ost_CN_42097854_380000_CN_54359256_380000/LConn1
  _CN_152261133_380000_CN_54359256_380000/RConn2 -- T_54359256_380000;220000;110000_Umspannwerk_Uchtelfangen/LConn2 -- _CN_54359256_380000_CN115145869/LConn2 -- 380_kV_Gilzem_Ost;_Uchtelfangen_Ost_CN_42097854_380000_CN_54359256_380000/LConn2
  _CN_152261133_380000_CN_54359256_380000/RConn3 -- T_54359256_380000;220000;110000_Umspannwerk_Uchtelfangen/LConn3 -- _CN_54359256_380000_CN115145869/LConn3 -- 380_kV_Gilzem_Ost;_Uchtelfangen_Ost_CN_42097854_380000_CN_54359256_380000/LConn3
  _CN_152261133_380000_CN_152018146_380000/RConn1 -- T_152018146_380000_Mittelbexbach/LConn1 -- _CN_152018146_380000_CN28051874/RConn1
  _CN_152261133_380000_CN_152018146_380000/RConn2 -- T_152018146_380000_Mittelbexbach/LConn2 -- _CN_152018146_380000_CN28051874/RConn2
  _CN_152261133_380000_CN_152018146_380000/RConn3 -- T_152018146_380000_Mittelbexbach/LConn3 -- _CN_152018146_380000_CN28051874/RConn3
  7563_CN_152261133_380000_CN_272646943_380000/RConn1 -- T_272646943_380000_/LConn1 -- 7563_CN_272646943_380000_CN152261126/LConn1
  7563_CN_152261133_380000_CN_272646943_380000/RConn2 -- T_272646943_380000_/LConn2 -- 7563_CN_272646943_380000_CN152261126/LConn2
  7563_CN_152261133_380000_CN_272646943_380000/RConn3 -- T_272646943_380000_/LConn3 -- 7563_CN_272646943_380000_CN152261126/LConn3
  T_194446360_380000_/LConn1 -- 7564_CN_152261133_380000_CN_194446360_380000/RConn1
  T_194446360_380000_/LConn2 -- 7564_CN_152261133_380000_CN_194446360_380000/RConn2
  T_194446360_380000_/LConn3 -- 7564_CN_152261133_380000_CN_194446360_380000/RConn3
  T_32966636_220000;110000_220_kV_Umspannwerk_Birkenfeld/LConn1 -- _CN_152261133_220000_CN_32966636_220000/RConn1
  T_32966636_220000;110000_220_kV_Umspannwerk_Birkenfeld/LConn2 -- _CN_152261133_220000_CN_32966636_220000/RConn2
  T_32966636_220000;110000_220_kV_Umspannwerk_Birkenfeld/LConn3 -- _CN_152261133_220000_CN_32966636_220000/RConn3
  _CN_152261133_220000_CN_32725957_220000/RConn1 -- T_32725957_220000;110000_Umspannwerk_Oberwald/LConn1 -- _CN_32725957_220000_CN_32725958_220000/LConn1
  _CN_152261133_220000_CN_32725957_220000/RConn2 -- T_32725957_220000;110000_Umspannwerk_Oberwald/LConn2 -- _CN_32725957_220000_CN_32725958_220000/LConn2
  _CN_152261133_220000_CN_32725957_220000/RConn3 -- T_32725957_220000;110000_Umspannwerk_Oberwald/LConn3 -- _CN_32725957_220000_CN_32725958_220000/LConn3
  _CN_242756113_220000_CN_87653464_220000/LConn1 -- T_242756113_380000;220000;110000_380_kV_Umspannwerk_Eichstetten/RConn1 -- L_242756113/LConn1
  _CN_242756113_220000_CN_87653464_220000/LConn2 -- T_242756113_380000;220000;110000_380_kV_Umspannwerk_Eichstetten/RConn2 -- L_242756113/LConn2
  _CN_242756113_220000_CN_87653464_220000/LConn3 -- T_242756113_380000;220000;110000_380_kV_Umspannwerk_Eichstetten/RConn3 -- L_242756113/LConn3
  _CN_242756113_220000_CN_87653464_220000/RConn1 -- T_87653464_220000;110000_220_kV_Umspannwerk_Eichstetten/LConn1 -- _CN_31367937_220000_CN_87653464_220000/LConn1 -- _CN_87653464_220000_CN_146962222_220000/RConn1
  _CN_242756113_220000_CN_87653464_220000/RConn2 -- T_87653464_220000;110000_220_kV_Umspannwerk_Eichstetten/LConn2 -- _CN_31367937_220000_CN_87653464_220000/LConn2 -- _CN_87653464_220000_CN_146962222_220000/RConn2
  _CN_242756113_220000_CN_87653464_220000/RConn3 -- T_87653464_220000;110000_220_kV_Umspannwerk_Eichstetten/LConn3 -- _CN_31367937_220000_CN_87653464_220000/LConn3 -- _CN_87653464_220000_CN_146962222_220000/RConn3
  380kV_Lippe_Süd_CN_23022100_380000_CN_24462426_380000/RConn1 -- T_24462426_380000;220000;110000_Station_Niederrhein/LConn1 -- _CN_24462426_380000_CN401873466/LConn1
  380kV_Lippe_Süd_CN_23022100_380000_CN_24462426_380000/RConn2 -- T_24462426_380000;220000;110000_Station_Niederrhein/LConn2 -- _CN_24462426_380000_CN401873466/LConn2
  380kV_Lippe_Süd_CN_23022100_380000_CN_24462426_380000/RConn3 -- T_24462426_380000;220000;110000_Station_Niederrhein/LConn3 -- _CN_24462426_380000_CN401873466/LConn3
  T_24280460_380000;110000_Station_Nordlicht/LConn1 -- 380kV_Kusenhorst_CN_23022100_380000_CN_24280460_380000/RConn1
  T_24280460_380000;110000_Station_Nordlicht/LConn2 -- 380kV_Kusenhorst_CN_23022100_380000_CN_24280460_380000/RConn2
  T_24280460_380000;110000_Station_Nordlicht/LConn3 -- 380kV_Kusenhorst_CN_23022100_380000_CN_24280460_380000/RConn3
  T_26291794_380000;110000_Station_Rosenblumendelle/LConn1 -- 380kV_Kusenhorst_CN_23022100_380000_CN_26291794_380000/RConn1
  T_26291794_380000;110000_Station_Rosenblumendelle/LConn2 -- 380kV_Kusenhorst_CN_23022100_380000_CN_26291794_380000/RConn2
  T_26291794_380000;110000_Station_Rosenblumendelle/LConn3 -- 380kV_Kusenhorst_CN_23022100_380000_CN_26291794_380000/RConn3
  T_24921206_380000;220000_Station_Büscherhof/LConn1 -- 380kV_Kusenhorst_CN_23022100_380000_CN_24921206_380000/RConn1
  T_24921206_380000;220000_Station_Büscherhof/LConn2 -- 380kV_Kusenhorst_CN_23022100_380000_CN_24921206_380000/RConn2
  T_24921206_380000;220000_Station_Büscherhof/LConn3 -- 380kV_Kusenhorst_CN_23022100_380000_CN_24921206_380000/RConn3
  _CN_30132758_380000_CN_43163132_380000/RConn1 -- T_43163132_380000;110000_Umspannwerk_Reuter/LConn1 -- _CN_43163132_380000_CN185569568/LConn1 -- 903;_904_CN_11500045_380000_CN_43163132_380000/LConn1
  _CN_30132758_380000_CN_43163132_380000/RConn2 -- T_43163132_380000;110000_Umspannwerk_Reuter/LConn2 -- _CN_43163132_380000_CN185569568/LConn2 -- 903;_904_CN_11500045_380000_CN_43163132_380000/LConn2
  _CN_30132758_380000_CN_43163132_380000/RConn3 -- T_43163132_380000;110000_Umspannwerk_Reuter/LConn3 -- _CN_43163132_380000_CN185569568/LConn3 -- 903;_904_CN_11500045_380000_CN_43163132_380000/LConn3
  T_78441561_380000;110000_Umspannwerk_Plattling/LConn1 -- Pleinting___Plattling___Schwandorf_CN_78441561_380000_CN_28956649_380000/LConn1
  T_78441561_380000;110000_Umspannwerk_Plattling/LConn2 -- Pleinting___Plattling___Schwandorf_CN_78441561_380000_CN_28956649_380000/LConn2
  T_78441561_380000;110000_Umspannwerk_Plattling/LConn3 -- Pleinting___Plattling___Schwandorf_CN_78441561_380000_CN_28956649_380000/LConn3
  Pleinting___Plattling___Schwandorf_CN_78441561_380000_CN_28956649_380000/RConn1 -- T_28956649_380000;220000;110000_Schwandorf/LConn1 -- Schwandorf___Etzenricht_CN_29084374_380000_CN_28956649_380000/RConn1
  Pleinting___Plattling___Schwandorf_CN_78441561_380000_CN_28956649_380000/RConn2 -- T_28956649_380000;220000;110000_Schwandorf/LConn2 -- Schwandorf___Etzenricht_CN_29084374_380000_CN_28956649_380000/RConn2
  Pleinting___Plattling___Schwandorf_CN_78441561_380000_CN_28956649_380000/RConn3 -- T_28956649_380000;220000;110000_Schwandorf/LConn3 -- Schwandorf___Etzenricht_CN_29084374_380000_CN_28956649_380000/RConn3
  G_129989100_Kavernenkraftwerk_Säckingen/RConn1 -- Öldruckkabel_CN_202865176_220000_CN129989100/RConn1
  G_129989100_Kavernenkraftwerk_Säckingen/RConn2 -- Öldruckkabel_CN_202865176_220000_CN129989100/RConn2
  G_129989100_Kavernenkraftwerk_Säckingen/RConn3 -- Öldruckkabel_CN_202865176_220000_CN129989100/RConn3
  T_24462228_220000;110000_Station_Ossenberg/LConn1 -- 220kV_Wesel_Ost_CN_24462426_220000_CN_24462228_220000/RConn1
  T_24462228_220000;110000_Station_Ossenberg/LConn2 -- 220kV_Wesel_Ost_CN_24462426_220000_CN_24462228_220000/RConn2
  T_24462228_220000;110000_Station_Ossenberg/LConn3 -- 220kV_Wesel_Ost_CN_24462426_220000_CN_24462228_220000/RConn3
  T_23084417_220000;110000_Station_Pfalzdorf/LConn1 -- _CN_24462426_220000_CN_23084417_220000/RConn1
  T_23084417_220000;110000_Station_Pfalzdorf/LConn2 -- _CN_24462426_220000_CN_23084417_220000/RConn2
  T_23084417_220000;110000_Station_Pfalzdorf/LConn3 -- _CN_24462426_220000_CN_23084417_220000/RConn3
  _CN_24462426_380000_CN401873466/RConn1 -- G_401873466_Kraftwerk_Voerde/RConn1 -- _CN_24479003_380000_CN401873466/LConn1 -- _CN_24479003_220000_CN401873466/LConn1 -- 380kV_Voerde_B_CN_76185022_380000_CN401873466/LConn1
  _CN_24462426_380000_CN401873466/RConn2 -- G_401873466_Kraftwerk_Voerde/RConn2 -- _CN_24479003_380000_CN401873466/LConn2 -- _CN_24479003_220000_CN401873466/LConn2 -- 380kV_Voerde_B_CN_76185022_380000_CN401873466/LConn2
  _CN_24462426_380000_CN401873466/RConn3 -- G_401873466_Kraftwerk_Voerde/RConn3 -- _CN_24479003_380000_CN401873466/LConn3 -- _CN_24479003_220000_CN401873466/LConn3 -- 380kV_Voerde_B_CN_76185022_380000_CN401873466/LConn3
  Leitung_2008_CN_33042984_220000_CN-2022229/RConn1 -- T_33042984_220000;110000_TenneT_TSO_GmbH___Betriebszentrum_Lehrte/LConn1 -- Leitung_2026_CN_33042984_220000_CN23681460/RConn1 -- _CN_33042984_220000_CN_160093341_220000/LConn1 -- _CN_33042984_220000_CN_43072656_220000/LConn1 -- _CN_33042984_220000_CN_30109913_220000/LConn1
  Leitung_2008_CN_33042984_220000_CN-2022229/RConn2 -- T_33042984_220000;110000_TenneT_TSO_GmbH___Betriebszentrum_Lehrte/LConn2 -- Leitung_2026_CN_33042984_220000_CN23681460/RConn2 -- _CN_33042984_220000_CN_160093341_220000/LConn2 -- _CN_33042984_220000_CN_43072656_220000/LConn2 -- _CN_33042984_220000_CN_30109913_220000/LConn2
  Leitung_2008_CN_33042984_220000_CN-2022229/RConn3 -- T_33042984_220000;110000_TenneT_TSO_GmbH___Betriebszentrum_Lehrte/LConn3 -- Leitung_2026_CN_33042984_220000_CN23681460/RConn3 -- _CN_33042984_220000_CN_160093341_220000/LConn3 -- _CN_33042984_220000_CN_43072656_220000/LConn3 -- _CN_33042984_220000_CN_30109913_220000/LConn3
  T_160093341_220000_Erzhausen/LConn1 -- _CN_33042984_220000_CN_160093341_220000/RConn1
  T_160093341_220000_Erzhausen/LConn2 -- _CN_33042984_220000_CN_160093341_220000/RConn2
  T_160093341_220000_Erzhausen/LConn3 -- _CN_33042984_220000_CN_160093341_220000/RConn3
  _CN_33042984_220000_CN_43072656_220000/RConn1 -- T_43072656_220000;110000_Hardegsen/LConn1 -- Leitung_2014_CN_43072656_220000_CN_29103809_220000/LConn1
  _CN_33042984_220000_CN_43072656_220000/RConn2 -- T_43072656_220000;110000_Hardegsen/LConn2 -- Leitung_2014_CN_43072656_220000_CN_29103809_220000/LConn2
  _CN_33042984_220000_CN_43072656_220000/RConn3 -- T_43072656_220000;110000_Hardegsen/LConn3 -- Leitung_2014_CN_43072656_220000_CN_29103809_220000/LConn3
  T_30109913_220000;110000_Godenau/LConn1 -- _CN_33042984_220000_CN_30109913_220000/RConn1
  T_30109913_220000;110000_Godenau/LConn2 -- _CN_33042984_220000_CN_30109913_220000/RConn2
  T_30109913_220000;110000_Godenau/LConn3 -- _CN_33042984_220000_CN_30109913_220000/RConn3
  T_202580524_380000_/LConn1 -- 380kV_Westfalen_D+E_CN_202580524_380000_CN_42488850_380000/RConn1
  T_202580524_380000_/LConn2 -- 380kV_Westfalen_D+E_CN_202580524_380000_CN_42488850_380000/RConn2
  T_202580524_380000_/LConn3 -- 380kV_Westfalen_D+E_CN_202580524_380000_CN_42488850_380000/RConn3
  G_31023006_/RConn1 -- _CN_88945213_380000_CN31023006/RConn1
  G_31023006_/RConn2 -- _CN_88945213_380000_CN31023006/RConn2
  G_31023006_/RConn3 -- _CN_88945213_380000_CN31023006/RConn3
  T_31019939_380000;110000_Gundremmingen/LConn1 -- _CN_88945213_380000_CN_31019939_380000/RConn1
  T_31019939_380000;110000_Gundremmingen/LConn2 -- _CN_88945213_380000_CN_31019939_380000/RConn2
  T_31019939_380000;110000_Gundremmingen/LConn3 -- _CN_88945213_380000_CN_31019939_380000/RConn3
  T_50643382_220000_Cloppenburg_220_kV/LConn1 -- 206_CN_50643382_220000_CN_173178563_220000/LConn1
  T_50643382_220000_Cloppenburg_220_kV/LConn2 -- 206_CN_50643382_220000_CN_173178563_220000/LConn2
  T_50643382_220000_Cloppenburg_220_kV/LConn3 -- 206_CN_50643382_220000_CN_173178563_220000/LConn3
  206_CN_50643382_220000_CN_173178563_220000/RConn1 -- T_173178563_220000;110000_Conneforde_110_220_kV/LConn1 -- 302_CN_32076853_220000_CN_173178563_220000/LConn1 -- 204_CN_173178563_220000_CN_23744346_220000/LConn1 -- 203_CN_34835258_220000_CN_173178563_220000/RConn1 -- Conneforde_220_kV_CN_23837631_220000_CN_173178563_220000/LConn1
  206_CN_50643382_220000_CN_173178563_220000/RConn2 -- T_173178563_220000;110000_Conneforde_110_220_kV/LConn2 -- 302_CN_32076853_220000_CN_173178563_220000/LConn2 -- 204_CN_173178563_220000_CN_23744346_220000/LConn2 -- 203_CN_34835258_220000_CN_173178563_220000/RConn2 -- Conneforde_220_kV_CN_23837631_220000_CN_173178563_220000/LConn2
  206_CN_50643382_220000_CN_173178563_220000/RConn3 -- T_173178563_220000;110000_Conneforde_110_220_kV/LConn3 -- 302_CN_32076853_220000_CN_173178563_220000/LConn3 -- 204_CN_173178563_220000_CN_23744346_220000/LConn3 -- 203_CN_34835258_220000_CN_173178563_220000/RConn3 -- Conneforde_220_kV_CN_23837631_220000_CN_173178563_220000/LConn3
  220_kV_Godorf_Ost;_Olefin_West_CN_22766160_220000_CN_32148946_220000/LConn1 -- T_22766160_380000;220000;110000_Station_Sechtem/RConn1 -- 220_kV_Troisdorf_West_CN_22766160_220000_CN_22767509_220000/RConn1 -- 220_kV_Knapsack_2b_CN_22766160_220000_CN_201153704_220000/LConn1 -- L_22766160/LConn1 -- 220_kV_Godorf_Ost;_Olefin_West_CN_22766160_220000_CN_23084554_220000/LConn1
  220_kV_Godorf_Ost;_Olefin_West_CN_22766160_220000_CN_32148946_220000/LConn2 -- T_22766160_380000;220000;110000_Station_Sechtem/RConn2 -- 220_kV_Troisdorf_West_CN_22766160_220000_CN_22767509_220000/RConn2 -- 220_kV_Knapsack_2b_CN_22766160_220000_CN_201153704_220000/LConn2 -- L_22766160/LConn2 -- 220_kV_Godorf_Ost;_Olefin_West_CN_22766160_220000_CN_23084554_220000/LConn2
  220_kV_Godorf_Ost;_Olefin_West_CN_22766160_220000_CN_32148946_220000/LConn3 -- T_22766160_380000;220000;110000_Station_Sechtem/RConn3 -- 220_kV_Troisdorf_West_CN_22766160_220000_CN_22767509_220000/RConn3 -- 220_kV_Knapsack_2b_CN_22766160_220000_CN_201153704_220000/LConn3 -- L_22766160/LConn3 -- 220_kV_Godorf_Ost;_Olefin_West_CN_22766160_220000_CN_23084554_220000/LConn3
  T_32148946_220000;110000_Station_Bollenacker/LConn1 -- 220_kV_Godorf_Ost;_Olefin_West_CN_22766160_220000_CN_32148946_220000/RConn1
  T_32148946_220000;110000_Station_Bollenacker/LConn2 -- 220_kV_Godorf_Ost;_Olefin_West_CN_22766160_220000_CN_32148946_220000/RConn2
  T_32148946_220000;110000_Station_Bollenacker/LConn3 -- 220_kV_Godorf_Ost;_Olefin_West_CN_22766160_220000_CN_32148946_220000/RConn3
  220_kV_Godorf_Ost;_Olefin_West_CN_22766160_220000_CN_23084554_220000/RConn1 -- T_23084554_220000;110000_Station_Brauweiler/LConn1 -- 220_kV_Bocklemünd_Nord|Süd_(Brauweiler)_CN_22690852_220000_CN_23084554_220000/LConn1 -- 220_kV_Rommerskirchen_Ost_CN_24839976_220000_CN_23084554_220000/RConn1
  220_kV_Godorf_Ost;_Olefin_West_CN_22766160_220000_CN_23084554_220000/RConn2 -- T_23084554_220000;110000_Station_Brauweiler/LConn2 -- 220_kV_Bocklemünd_Nord|Süd_(Brauweiler)_CN_22690852_220000_CN_23084554_220000/LConn2 -- 220_kV_Rommerskirchen_Ost_CN_24839976_220000_CN_23084554_220000/RConn2
  220_kV_Godorf_Ost;_Olefin_West_CN_22766160_220000_CN_23084554_220000/RConn3 -- T_23084554_220000;110000_Station_Brauweiler/LConn3 -- 220_kV_Bocklemünd_Nord|Süd_(Brauweiler)_CN_22690852_220000_CN_23084554_220000/LConn3 -- 220_kV_Rommerskirchen_Ost_CN_24839976_220000_CN_23084554_220000/RConn3
  380_kV_Siegtal_Nord|Süd_CN_22766160_380000_CN_152403632_380000/RConn1 -- T_22766160_380000;220000;110000_Station_Sechtem/LConn1 -- 380_kV_Sechtem_Nord|Süd;_Walberberg_West_CN_22766160_380000_CN_26593929_380000/RConn1 -- 380_kV_Ville_Ost_CN_22766160_380000_CN_22765517_380000/LConn1 -- 380_kV_Ville_Ost_CN_22766160_380000_CN_24839976_380000/RConn1 -- 380_kV_Liessem_Ost;Mittelrhein_CN_22766160_380000_CN_395847307_380000/LConn1 -- 380_kV_Liessem_Ost;Mittelrhein_CN_22766160_380000_CN_26777313_380000/LConn1
  380_kV_Siegtal_Nord|Süd_CN_22766160_380000_CN_152403632_380000/RConn2 -- T_22766160_380000;220000;110000_Station_Sechtem/LConn2 -- 380_kV_Sechtem_Nord|Süd;_Walberberg_West_CN_22766160_380000_CN_26593929_380000/RConn2 -- 380_kV_Ville_Ost_CN_22766160_380000_CN_22765517_380000/LConn2 -- 380_kV_Ville_Ost_CN_22766160_380000_CN_24839976_380000/RConn2 -- 380_kV_Liessem_Ost;Mittelrhein_CN_22766160_380000_CN_395847307_380000/LConn2 -- 380_kV_Liessem_Ost;Mittelrhein_CN_22766160_380000_CN_26777313_380000/LConn2
  380_kV_Siegtal_Nord|Süd_CN_22766160_380000_CN_152403632_380000/RConn3 -- T_22766160_380000;220000;110000_Station_Sechtem/LConn3 -- 380_kV_Sechtem_Nord|Süd;_Walberberg_West_CN_22766160_380000_CN_26593929_380000/RConn3 -- 380_kV_Ville_Ost_CN_22766160_380000_CN_22765517_380000/LConn3 -- 380_kV_Ville_Ost_CN_22766160_380000_CN_24839976_380000/RConn3 -- 380_kV_Liessem_Ost;Mittelrhein_CN_22766160_380000_CN_395847307_380000/LConn3 -- 380_kV_Liessem_Ost;Mittelrhein_CN_22766160_380000_CN_26777313_380000/LConn3
  380_kV_Ville_Ost_CN_22766160_380000_CN_22765517_380000/RConn1 -- T_22765517_380000;110000_Station_Knapsack/LConn1 -- _CN_22765517_380000_CN239364386/LConn1 -- 380_kV_Knapsack_1a_CN_201153704_380000_CN_22765517_380000/LConn1
  380_kV_Ville_Ost_CN_22766160_380000_CN_22765517_380000/RConn2 -- T_22765517_380000;110000_Station_Knapsack/LConn2 -- _CN_22765517_380000_CN239364386/LConn2 -- 380_kV_Knapsack_1a_CN_201153704_380000_CN_22765517_380000/LConn2
  380_kV_Ville_Ost_CN_22766160_380000_CN_22765517_380000/RConn3 -- T_22765517_380000;110000_Station_Knapsack/LConn3 -- _CN_22765517_380000_CN239364386/LConn3 -- 380_kV_Knapsack_1a_CN_201153704_380000_CN_22765517_380000/LConn3
  380_kV_Liessem_Ost;Mittelrhein_CN_22766160_380000_CN_395847307_380000/RConn1 -- T_395847307_380000;220000;110000_Station_Weißenthurm/LConn1 -- _CN_160584794_380000_CN_395847307_380000/LConn1
  380_kV_Liessem_Ost;Mittelrhein_CN_22766160_380000_CN_395847307_380000/RConn2 -- T_395847307_380000;220000;110000_Station_Weißenthurm/LConn2 -- _CN_160584794_380000_CN_395847307_380000/LConn2
  380_kV_Liessem_Ost;Mittelrhein_CN_22766160_380000_CN_395847307_380000/RConn3 -- T_395847307_380000;220000;110000_Station_Weißenthurm/LConn3 -- _CN_160584794_380000_CN_395847307_380000/LConn3
  T_26777313_380000;110000_Station_Ließem/LConn1 -- 380_kV_Liessem_Ost;Mittelrhein_CN_22766160_380000_CN_26777313_380000/RConn1
  T_26777313_380000;110000_Station_Ließem/LConn2 -- 380_kV_Liessem_Ost;Mittelrhein_CN_22766160_380000_CN_26777313_380000/RConn2
  T_26777313_380000;110000_Station_Ließem/LConn3 -- 380_kV_Liessem_Ost;Mittelrhein_CN_22766160_380000_CN_26777313_380000/RConn3
  220_kV_Knapsack_2b_CN_22766160_220000_CN_201153704_220000/RConn1 -- T_201153704_380000;220000_Kraftwerkschaltanlage_Knapsack_1/RConn1 -- L_201153704/LConn1
  220_kV_Knapsack_2b_CN_22766160_220000_CN_201153704_220000/RConn2 -- T_201153704_380000;220000_Kraftwerkschaltanlage_Knapsack_1/RConn2 -- L_201153704/LConn2
  220_kV_Knapsack_2b_CN_22766160_220000_CN_201153704_220000/RConn3 -- T_201153704_380000;220000_Kraftwerkschaltanlage_Knapsack_1/RConn3 -- L_201153704/LConn3
  EDS_WDL_1x_380_kV_CN_26260052_380000_CN_26403575_380000/LConn1 -- T_26260052_380000;220000;110000_EnBW_Umspannwerk_Wendlingen/LConn1 -- EDS_WDL_1x_380_kV_CN_26260052_380000_CN_30734324_380000/LConn1 -- EDS_WDL_1x_380_kV_CN_26260052_380000_CN25973419/LConn1 -- 380_kV_CN_26260052_380000_CN_25802269_380000/LConn1 -- 380_kV_CN_26260052_380000_CN_43688805_380000/RConn1 -- 380_kV_CN_26260052_380000_CN_22960899_380000/LConn1 -- 380_kV_CN_26260052_380000_CN_41389594_380000/RConn1
  EDS_WDL_1x_380_kV_CN_26260052_380000_CN_26403575_380000/LConn2 -- T_26260052_380000;220000;110000_EnBW_Umspannwerk_Wendlingen/LConn2 -- EDS_WDL_1x_380_kV_CN_26260052_380000_CN_30734324_380000/LConn2 -- EDS_WDL_1x_380_kV_CN_26260052_380000_CN25973419/LConn2 -- 380_kV_CN_26260052_380000_CN_25802269_380000/LConn2 -- 380_kV_CN_26260052_380000_CN_43688805_380000/RConn2 -- 380_kV_CN_26260052_380000_CN_22960899_380000/LConn2 -- 380_kV_CN_26260052_380000_CN_41389594_380000/RConn2
  EDS_WDL_1x_380_kV_CN_26260052_380000_CN_26403575_380000/LConn3 -- T_26260052_380000;220000;110000_EnBW_Umspannwerk_Wendlingen/LConn3 -- EDS_WDL_1x_380_kV_CN_26260052_380000_CN_30734324_380000/LConn3 -- EDS_WDL_1x_380_kV_CN_26260052_380000_CN25973419/LConn3 -- 380_kV_CN_26260052_380000_CN_25802269_380000/LConn3 -- 380_kV_CN_26260052_380000_CN_43688805_380000/RConn3 -- 380_kV_CN_26260052_380000_CN_22960899_380000/LConn3 -- 380_kV_CN_26260052_380000_CN_41389594_380000/RConn3
  T_26403575_380000;110000_EnBW_Umspannwerk_Bünzwangen/LConn1 -- EDS_WDL_1x_380_kV_CN_26260052_380000_CN_26403575_380000/RConn1
  T_26403575_380000;110000_EnBW_Umspannwerk_Bünzwangen/LConn2 -- EDS_WDL_1x_380_kV_CN_26260052_380000_CN_26403575_380000/RConn2
  T_26403575_380000;110000_EnBW_Umspannwerk_Bünzwangen/LConn3 -- EDS_WDL_1x_380_kV_CN_26260052_380000_CN_26403575_380000/RConn3
  T_30734324_380000;220000;110000_EnBW_Umspannwerk_Metzingen/LConn1 -- EDS_WDL_1x_380_kV_CN_26260052_380000_CN_30734324_380000/RConn1
  T_30734324_380000;220000;110000_EnBW_Umspannwerk_Metzingen/LConn2 -- EDS_WDL_1x_380_kV_CN_26260052_380000_CN_30734324_380000/RConn2
  T_30734324_380000;220000;110000_EnBW_Umspannwerk_Metzingen/LConn3 -- EDS_WDL_1x_380_kV_CN_26260052_380000_CN_30734324_380000/RConn3
  EDS_WDL_1x_380_kV_CN_26260052_380000_CN25973419/RConn1 -- G_25973419_Heizkraftwerk_Altbach_Deizisau/RConn1 -- AL1_EDS_380_kV_CN_48428875_380000_CN25973419/LConn1 -- AL1_BZW_380_kV_CN_37721677_380000_CN25973419/LConn1
  EDS_WDL_1x_380_kV_CN_26260052_380000_CN25973419/RConn2 -- G_25973419_Heizkraftwerk_Altbach_Deizisau/RConn2 -- AL1_EDS_380_kV_CN_48428875_380000_CN25973419/LConn2 -- AL1_BZW_380_kV_CN_37721677_380000_CN25973419/LConn2
  EDS_WDL_1x_380_kV_CN_26260052_380000_CN25973419/RConn3 -- G_25973419_Heizkraftwerk_Altbach_Deizisau/RConn3 -- AL1_EDS_380_kV_CN_48428875_380000_CN25973419/LConn3 -- AL1_BZW_380_kV_CN_37721677_380000_CN25973419/LConn3
  380_kV_CN_26260052_380000_CN_25802269_380000/RConn1 -- T_25802269_380000;220000;110000_Umspannstation_Hoheneck_Amprion/LConn1 -- _CN_25802269_380000_CN_149987048_380000/RConn1
  380_kV_CN_26260052_380000_CN_25802269_380000/RConn2 -- T_25802269_380000;220000;110000_Umspannstation_Hoheneck_Amprion/LConn2 -- _CN_25802269_380000_CN_149987048_380000/RConn2
  380_kV_CN_26260052_380000_CN_25802269_380000/RConn3 -- T_25802269_380000;220000;110000_Umspannstation_Hoheneck_Amprion/LConn3 -- _CN_25802269_380000_CN_149987048_380000/RConn3
  T_22960899_380000;110000_Umspannwerk_Mühlhausen/LConn1 -- 380_kV_CN_26260052_380000_CN_22960899_380000/RConn1
  T_22960899_380000;110000_Umspannwerk_Mühlhausen/LConn2 -- 380_kV_CN_26260052_380000_CN_22960899_380000/RConn2
  T_22960899_380000;110000_Umspannwerk_Mühlhausen/LConn3 -- 380_kV_CN_26260052_380000_CN_22960899_380000/RConn3
  T_59026005_380000;110000_Umspannwerk_Hagenwerder/LConn1 -- _CN_59026005_380000_CN_157807291_380000/RConn1
  T_59026005_380000;110000_Umspannwerk_Hagenwerder/LConn2 -- _CN_59026005_380000_CN_157807291_380000/RConn2
  T_59026005_380000;110000_Umspannwerk_Hagenwerder/LConn3 -- _CN_59026005_380000_CN_157807291_380000/RConn3
  220kV_Siegerland_West_CN_89043564_220000_CN_132814303_220000/RConn1 -- T_89043564_220000;110000_Station_Eiserfeld/LConn1 -- 220kV_Siegerland_West_CN_89043564_220000_CN_152403632_220000/LConn1
  220kV_Siegerland_West_CN_89043564_220000_CN_132814303_220000/RConn2 -- T_89043564_220000;110000_Station_Eiserfeld/LConn2 -- 220kV_Siegerland_West_CN_89043564_220000_CN_152403632_220000/LConn2
  220kV_Siegerland_West_CN_89043564_220000_CN_132814303_220000/RConn3 -- T_89043564_220000;110000_Station_Eiserfeld/LConn3 -- 220kV_Siegerland_West_CN_89043564_220000_CN_152403632_220000/LConn3
  220kV_Siegerland_West_CN_89043564_220000_CN_152403632_220000/RConn1 -- T_152403632_380000;220000;110000_Station_Dauersberg/RConn1 -- 220_kV_Leuscheid_Nord+Süd_CN_152403632_220000_CN_22767509_220000/RConn1 -- L_152403632/LConn1
  220kV_Siegerland_West_CN_89043564_220000_CN_152403632_220000/RConn2 -- T_152403632_380000;220000;110000_Station_Dauersberg/RConn2 -- 220_kV_Leuscheid_Nord+Süd_CN_152403632_220000_CN_22767509_220000/RConn2 -- L_152403632/LConn2
  220kV_Siegerland_West_CN_89043564_220000_CN_152403632_220000/RConn3 -- T_152403632_380000;220000;110000_Station_Dauersberg/RConn3 -- 220_kV_Leuscheid_Nord+Süd_CN_152403632_220000_CN_22767509_220000/RConn3 -- L_152403632/LConn3
  PULVE_OBJTT_ENGST_380_kV;_OBJTT_ENGST_380_kV;_TRSNG_WDLNG_220_kV_CN_42736239_380000_CN_26814283_380000/RConn1 -- T_26814283_380000;110000_EnBW_Umspannwerk_Oberjettingen/LConn1 -- 2x_380_kV_CN_43688805_380000_CN_26814283_380000/RConn1
  PULVE_OBJTT_ENGST_380_kV;_OBJTT_ENGST_380_kV;_TRSNG_WDLNG_220_kV_CN_42736239_380000_CN_26814283_380000/RConn2 -- T_26814283_380000;110000_EnBW_Umspannwerk_Oberjettingen/LConn2 -- 2x_380_kV_CN_43688805_380000_CN_26814283_380000/RConn2
  PULVE_OBJTT_ENGST_380_kV;_OBJTT_ENGST_380_kV;_TRSNG_WDLNG_220_kV_CN_42736239_380000_CN_26814283_380000/RConn3 -- T_26814283_380000;110000_EnBW_Umspannwerk_Oberjettingen/LConn3 -- 2x_380_kV_CN_43688805_380000_CN_26814283_380000/RConn3
  2_x_380_kV;_3_x_220_kV_CN_23284340_220000_CN_160533153_220000/LConn1 -- T_23284340_380000;220000;110000_Umspannwerk_Urberach/RConn1 -- 2_x_380_kV;_3_x_220_kV_CN_23284340_220000_CN_274609757_220000/LConn1 -- L_23284340/LConn1
  2_x_380_kV;_3_x_220_kV_CN_23284340_220000_CN_160533153_220000/LConn2 -- T_23284340_380000;220000;110000_Umspannwerk_Urberach/RConn2 -- 2_x_380_kV;_3_x_220_kV_CN_23284340_220000_CN_274609757_220000/LConn2 -- L_23284340/LConn2
  2_x_380_kV;_3_x_220_kV_CN_23284340_220000_CN_160533153_220000/LConn3 -- T_23284340_380000;220000;110000_Umspannwerk_Urberach/RConn3 -- 2_x_380_kV;_3_x_220_kV_CN_23284340_220000_CN_274609757_220000/LConn3 -- L_23284340/LConn3
  T_160533153_220000;110000_Beerfelden/LConn1 -- 2_x_380_kV;_3_x_220_kV_CN_23284340_220000_CN_160533153_220000/RConn1
  T_160533153_220000;110000_Beerfelden/LConn2 -- 2_x_380_kV;_3_x_220_kV_CN_23284340_220000_CN_160533153_220000/RConn2
  T_160533153_220000;110000_Beerfelden/LConn3 -- 2_x_380_kV;_3_x_220_kV_CN_23284340_220000_CN_160533153_220000/RConn3
  2_x_380_kV;_3_x_220_kV_CN_23284340_380000_CN_24685992_380000/LConn1 -- T_23284340_380000;220000;110000_Umspannwerk_Urberach/LConn1 -- 380_kV_CN_23284340_380000_CN_42372159_380000/LConn1 -- 380_kV_CN_23284340_380000_CN_42410916_380000/LConn1 -- 2_x_380_kV;_3_x_220_kV_CN_23284340_380000_CN_55730023_380000/RConn1 -- 2_x_380_kV;_3_x_220_kV_CN_23284340_380000_CN_160584794_380000/LConn1 -- 2_x_380_kV;_3_x_220_kV_CN_23284340_380000_CN_50898216_380000/LConn1 -- 2_x_380_kV;_3_x_220_kV_CN_23284340_380000_CN_38661452_380000/LConn1 -- 2_x_380_kV;_3_x_220_kV_CN_23284340_380000_CN_149987048_380000/RConn1 -- 2_x_380_kV;_3_x_220_kV_CN_23284340_380000_CN155389593/LConn1 -- 2_x_380_kV;_3_x_220_kV_CN_23284340_380000_CN_274609757_380000/LConn1
  2_x_380_kV;_3_x_220_kV_CN_23284340_380000_CN_24685992_380000/LConn2 -- T_23284340_380000;220000;110000_Umspannwerk_Urberach/LConn2 -- 380_kV_CN_23284340_380000_CN_42372159_380000/LConn2 -- 380_kV_CN_23284340_380000_CN_42410916_380000/LConn2 -- 2_x_380_kV;_3_x_220_kV_CN_23284340_380000_CN_55730023_380000/RConn2 -- 2_x_380_kV;_3_x_220_kV_CN_23284340_380000_CN_160584794_380000/LConn2 -- 2_x_380_kV;_3_x_220_kV_CN_23284340_380000_CN_50898216_380000/LConn2 -- 2_x_380_kV;_3_x_220_kV_CN_23284340_380000_CN_38661452_380000/LConn2 -- 2_x_380_kV;_3_x_220_kV_CN_23284340_380000_CN_149987048_380000/RConn2 -- 2_x_380_kV;_3_x_220_kV_CN_23284340_380000_CN155389593/LConn2 -- 2_x_380_kV;_3_x_220_kV_CN_23284340_380000_CN_274609757_380000/LConn2
  2_x_380_kV;_3_x_220_kV_CN_23284340_380000_CN_24685992_380000/LConn3 -- T_23284340_380000;220000;110000_Umspannwerk_Urberach/LConn3 -- 380_kV_CN_23284340_380000_CN_42372159_380000/LConn3 -- 380_kV_CN_23284340_380000_CN_42410916_380000/LConn3 -- 2_x_380_kV;_3_x_220_kV_CN_23284340_380000_CN_55730023_380000/RConn3 -- 2_x_380_kV;_3_x_220_kV_CN_23284340_380000_CN_160584794_380000/LConn3 -- 2_x_380_kV;_3_x_220_kV_CN_23284340_380000_CN_50898216_380000/LConn3 -- 2_x_380_kV;_3_x_220_kV_CN_23284340_380000_CN_38661452_380000/LConn3 -- 2_x_380_kV;_3_x_220_kV_CN_23284340_380000_CN_149987048_380000/RConn3 -- 2_x_380_kV;_3_x_220_kV_CN_23284340_380000_CN155389593/LConn3 -- 2_x_380_kV;_3_x_220_kV_CN_23284340_380000_CN_274609757_380000/LConn3
  T_24685992_380000;110000_Umspannstation_Bischofsheim/LConn1 -- 2_x_380_kV;_3_x_220_kV_CN_23284340_380000_CN_24685992_380000/RConn1
  T_24685992_380000;110000_Umspannstation_Bischofsheim/LConn2 -- 2_x_380_kV;_3_x_220_kV_CN_23284340_380000_CN_24685992_380000/RConn2
  T_24685992_380000;110000_Umspannstation_Bischofsheim/LConn3 -- 2_x_380_kV;_3_x_220_kV_CN_23284340_380000_CN_24685992_380000/RConn3
  2_x_380_kV;_3_x_220_kV_CN_23284340_380000_CN_160584794_380000/RConn1 -- T_160584794_380000;110000_Station_Koblenz/LConn1 -- _CN_160584794_380000_CN_395847307_380000/RConn1 -- _CN_160584794_380000_CN_149987048_380000/RConn1
  2_x_380_kV;_3_x_220_kV_CN_23284340_380000_CN_160584794_380000/RConn2 -- T_160584794_380000;110000_Station_Koblenz/LConn2 -- _CN_160584794_380000_CN_395847307_380000/RConn2 -- _CN_160584794_380000_CN_149987048_380000/RConn2
  2_x_380_kV;_3_x_220_kV_CN_23284340_380000_CN_160584794_380000/RConn3 -- T_160584794_380000;110000_Station_Koblenz/LConn3 -- _CN_160584794_380000_CN_395847307_380000/RConn3 -- _CN_160584794_380000_CN_149987048_380000/RConn3
  2_x_380_kV;_3_x_220_kV_CN_23284340_380000_CN_50898216_380000/RConn1 -- T_50898216_380000;110000_Station_Limburg/LConn1 -- 380kV_Limburg_West_CN_50898216_380000_CN_152403632_380000/RConn1
  2_x_380_kV;_3_x_220_kV_CN_23284340_380000_CN_50898216_380000/RConn2 -- T_50898216_380000;110000_Station_Limburg/LConn2 -- 380kV_Limburg_West_CN_50898216_380000_CN_152403632_380000/RConn2
  2_x_380_kV;_3_x_220_kV_CN_23284340_380000_CN_50898216_380000/RConn3 -- T_50898216_380000;110000_Station_Limburg/LConn3 -- 380kV_Limburg_West_CN_50898216_380000_CN_152403632_380000/RConn3
  T_38661452_380000;110000_Umspannwerk_Kriftel/LConn1 -- 2_x_380_kV;_3_x_220_kV_CN_23284340_380000_CN_38661452_380000/RConn1
  T_38661452_380000;110000_Umspannwerk_Kriftel/LConn2 -- 2_x_380_kV;_3_x_220_kV_CN_23284340_380000_CN_38661452_380000/RConn2
  T_38661452_380000;110000_Umspannwerk_Kriftel/LConn3 -- 2_x_380_kV;_3_x_220_kV_CN_23284340_380000_CN_38661452_380000/RConn3
  2_x_380_kV;_3_x_220_kV_CN_23284340_220000_CN_274609757_220000/RConn1 -- T_274609757_380000;220000_Biblis_A/RConn1 -- L_274609757/LConn1
  2_x_380_kV;_3_x_220_kV_CN_23284340_220000_CN_274609757_220000/RConn2 -- T_274609757_380000;220000_Biblis_A/RConn2 -- L_274609757/LConn2
  2_x_380_kV;_3_x_220_kV_CN_23284340_220000_CN_274609757_220000/RConn3 -- T_274609757_380000;220000_Biblis_A/RConn3 -- L_274609757/LConn3
  G_155389593_Kernkraftwerk_Biblis/RConn1 -- 2_x_380_kV;_3_x_220_kV_CN_23284340_380000_CN155389593/RConn1
  G_155389593_Kernkraftwerk_Biblis/RConn2 -- 2_x_380_kV;_3_x_220_kV_CN_23284340_380000_CN155389593/RConn2
  G_155389593_Kernkraftwerk_Biblis/RConn3 -- 2_x_380_kV;_3_x_220_kV_CN_23284340_380000_CN155389593/RConn3
  T_274609757_380000;220000_Biblis_A/LConn1 -- 2_x_380_kV;_3_x_220_kV_CN_23284340_380000_CN_274609757_380000/RConn1
  T_274609757_380000;220000_Biblis_A/LConn2 -- 2_x_380_kV;_3_x_220_kV_CN_23284340_380000_CN_274609757_380000/RConn2
  T_274609757_380000;220000_Biblis_A/LConn3 -- 2_x_380_kV;_3_x_220_kV_CN_23284340_380000_CN_274609757_380000/RConn3
  T_42372159_380000;110000_Karlstein/LConn1 -- 380_kV_CN_23284340_380000_CN_42372159_380000/RConn1
  T_42372159_380000;110000_Karlstein/LConn2 -- 380_kV_CN_23284340_380000_CN_42372159_380000/RConn2
  T_42372159_380000;110000_Karlstein/LConn3 -- 380_kV_CN_23284340_380000_CN_42372159_380000/RConn3
  380_kV_CN_23284340_380000_CN_42410916_380000/RConn1 -- T_42410916_380000;220000_Umspannwerk_Großkrotzenburg/LConn1 -- AS_GKRO;GKRO_GR_I;DIP_GKB_I;_II_CN_42410916_380000_CN_55069713_380000/LConn1 -- AS_GKRO;GKRO_GR_I;DIP_GKB_I;_II_CN_42410916_380000_CN_108797675_380000/RConn1 -- AS_GKRO;GKRO_GR_I;DIP_GKB_I;_II_CN_42410916_380000_CN_148446247_380000/LConn1 -- _CN_24042358_380000_CN_42410916_380000/LConn1
  380_kV_CN_23284340_380000_CN_42410916_380000/RConn2 -- T_42410916_380000;220000_Umspannwerk_Großkrotzenburg/LConn2 -- AS_GKRO;GKRO_GR_I;DIP_GKB_I;_II_CN_42410916_380000_CN_55069713_380000/LConn2 -- AS_GKRO;GKRO_GR_I;DIP_GKB_I;_II_CN_42410916_380000_CN_108797675_380000/RConn2 -- AS_GKRO;GKRO_GR_I;DIP_GKB_I;_II_CN_42410916_380000_CN_148446247_380000/LConn2 -- _CN_24042358_380000_CN_42410916_380000/LConn2
  380_kV_CN_23284340_380000_CN_42410916_380000/RConn3 -- T_42410916_380000;220000_Umspannwerk_Großkrotzenburg/LConn3 -- AS_GKRO;GKRO_GR_I;DIP_GKB_I;_II_CN_42410916_380000_CN_55069713_380000/LConn3 -- AS_GKRO;GKRO_GR_I;DIP_GKB_I;_II_CN_42410916_380000_CN_108797675_380000/RConn3 -- AS_GKRO;GKRO_GR_I;DIP_GKB_I;_II_CN_42410916_380000_CN_148446247_380000/LConn3 -- _CN_24042358_380000_CN_42410916_380000/LConn3
  T_274621059_220000;110000_Mehrum_(220_kV)/LConn1 -- Salzgitter_Hallendorf_CN_274621059_220000_CN23681460/RConn1
  T_274621059_220000;110000_Mehrum_(220_kV)/LConn2 -- Salzgitter_Hallendorf_CN_274621059_220000_CN23681460/RConn2
  T_274621059_220000;110000_Mehrum_(220_kV)/LConn3 -- Salzgitter_Hallendorf_CN_274621059_220000_CN23681460/RConn3
  T_46584363_380000;220000;110000_Umspannwerk_Wiesloch/LConn1 -- Elsenz_CN_143903369_380000_CN_46584363_380000/RConn1
  T_46584363_380000;220000;110000_Umspannwerk_Wiesloch/LConn2 -- Elsenz_CN_143903369_380000_CN_46584363_380000/RConn2
  T_46584363_380000;220000;110000_Umspannwerk_Wiesloch/LConn3 -- Elsenz_CN_143903369_380000_CN_46584363_380000/RConn3
  T_207248812_380000;220000_Umspannwerk_Neurott/LConn1 -- Elsenz_CN_143903369_380000_CN_207248812_380000/RConn1
  T_207248812_380000;220000_Umspannwerk_Neurott/LConn2 -- Elsenz_CN_143903369_380000_CN_207248812_380000/RConn2
  T_207248812_380000;220000_Umspannwerk_Neurott/LConn3 -- Elsenz_CN_143903369_380000_CN_207248812_380000/RConn3
  380kV_Mengede_Nord+Süd_CN_121199242_380000_CN109504648/LConn1 -- T_121199242_380000_Station_Lippe/LConn1 -- 380kV_Waltrop_Süd_CN_121199242_380000_CN4670340/LConn1 -- 380kV_Waltrop_Süd_CN_121199242_380000_CN_42507488_380000/RConn1 -- 380kV_Stummhafen_1A_CN_121199242_380000_CN109505608/LConn1 -- 380kV_Mengede_Nord+Süd_CN_121199242_380000_CN_32472806_380000/RConn1
  380kV_Mengede_Nord+Süd_CN_121199242_380000_CN109504648/LConn2 -- T_121199242_380000_Station_Lippe/LConn2 -- 380kV_Waltrop_Süd_CN_121199242_380000_CN4670340/LConn2 -- 380kV_Waltrop_Süd_CN_121199242_380000_CN_42507488_380000/RConn2 -- 380kV_Stummhafen_1A_CN_121199242_380000_CN109505608/LConn2 -- 380kV_Mengede_Nord+Süd_CN_121199242_380000_CN_32472806_380000/RConn2
  380kV_Mengede_Nord+Süd_CN_121199242_380000_CN109504648/LConn3 -- T_121199242_380000_Station_Lippe/LConn3 -- 380kV_Waltrop_Süd_CN_121199242_380000_CN4670340/LConn3 -- 380kV_Waltrop_Süd_CN_121199242_380000_CN_42507488_380000/RConn3 -- 380kV_Stummhafen_1A_CN_121199242_380000_CN109505608/LConn3 -- 380kV_Mengede_Nord+Süd_CN_121199242_380000_CN_32472806_380000/RConn3
  380kV_Mengede_Nord+Süd_CN_121199242_380000_CN109504648/RConn1 -- G_109504648_Kraftwerk_Datteln_4/RConn1 -- _CN_275138524_380000_CN109504648/LConn1
  380kV_Mengede_Nord+Süd_CN_121199242_380000_CN109504648/RConn2 -- G_109504648_Kraftwerk_Datteln_4/RConn2 -- _CN_275138524_380000_CN109504648/LConn2
  380kV_Mengede_Nord+Süd_CN_121199242_380000_CN109504648/RConn3 -- G_109504648_Kraftwerk_Datteln_4/RConn3 -- _CN_275138524_380000_CN109504648/LConn3
  G_4670340_Kraftwerk_Bergkamen/RConn1 -- 380kV_Waltrop_Süd_CN_121199242_380000_CN4670340/RConn1
  G_4670340_Kraftwerk_Bergkamen/RConn2 -- 380kV_Waltrop_Süd_CN_121199242_380000_CN4670340/RConn2
  G_4670340_Kraftwerk_Bergkamen/RConn3 -- 380kV_Waltrop_Süd_CN_121199242_380000_CN4670340/RConn3
  G_109505608_Trianel_Kraftwerk_Lünen/RConn1 -- 380kV_Stummhafen_1A_CN_121199242_380000_CN109505608/RConn1
  G_109505608_Trianel_Kraftwerk_Lünen/RConn2 -- 380kV_Stummhafen_1A_CN_121199242_380000_CN109505608/RConn2
  G_109505608_Trianel_Kraftwerk_Lünen/RConn3 -- 380kV_Stummhafen_1A_CN_121199242_380000_CN109505608/RConn3
  _CN_22973070_380000_CN_30954714_380000/RConn1 -- T_30954714_380000;110000_Umspannwerk_Friedrichshain/LConn1 -- 380_kV_Transversale_Berlin_CN_30954714_380000_CN_30303506_380000/LConn1
  _CN_22973070_380000_CN_30954714_380000/RConn2 -- T_30954714_380000;110000_Umspannwerk_Friedrichshain/LConn2 -- 380_kV_Transversale_Berlin_CN_30954714_380000_CN_30303506_380000/LConn2
  _CN_22973070_380000_CN_30954714_380000/RConn3 -- T_30954714_380000;110000_Umspannwerk_Friedrichshain/LConn3 -- 380_kV_Transversale_Berlin_CN_30954714_380000_CN_30303506_380000/LConn3
  T_26593935_380000_Station_Hambach/LConn1 -- _CN_26593935_380000_CN_26593929_380000/RConn1
  T_26593935_380000_Station_Hambach/LConn2 -- _CN_26593935_380000_CN_26593929_380000/RConn2
  T_26593935_380000_Station_Hambach/LConn3 -- _CN_26593935_380000_CN_26593929_380000/RConn3
  220kV_Neurath_1a+Osterath_West_CN_24799890_220000_CN_27919734_220000/RConn1 -- T_27919734_220000;110000_Station_Gohrpunkt/LConn1 -- 220_kV_Neurath_1a_CN_27919734_220000_CN_95434457_220000/LConn1 -- 220_kV_Neurath_1a_CN_27919734_220000_CN24267119/RConn1 -- 220_kV_Frixheim_Süd;_Zons_Nord_CN_27919734_220000_CN_49577401_220000/RConn1 -- 220_kV_Frixheim_Nord|Süd_CN_24839976_220000_CN_27919734_220000/RConn1
  220kV_Neurath_1a+Osterath_West_CN_24799890_220000_CN_27919734_220000/RConn2 -- T_27919734_220000;110000_Station_Gohrpunkt/LConn2 -- 220_kV_Neurath_1a_CN_27919734_220000_CN_95434457_220000/LConn2 -- 220_kV_Neurath_1a_CN_27919734_220000_CN24267119/RConn2 -- 220_kV_Frixheim_Süd;_Zons_Nord_CN_27919734_220000_CN_49577401_220000/RConn2 -- 220_kV_Frixheim_Nord|Süd_CN_24839976_220000_CN_27919734_220000/RConn2
  220kV_Neurath_1a+Osterath_West_CN_24799890_220000_CN_27919734_220000/RConn3 -- T_27919734_220000;110000_Station_Gohrpunkt/LConn3 -- 220_kV_Neurath_1a_CN_27919734_220000_CN_95434457_220000/LConn3 -- 220_kV_Neurath_1a_CN_27919734_220000_CN24267119/RConn3 -- 220_kV_Frixheim_Süd;_Zons_Nord_CN_27919734_220000_CN_49577401_220000/RConn3 -- 220_kV_Frixheim_Nord|Süd_CN_24839976_220000_CN_27919734_220000/RConn3
  T_35818134_220000;110000_Station_Ruhrort/LConn1 -- Stockum_Ost+West_CN_35818134_220000_CN_35818137_220000/RConn1
  T_35818134_220000;110000_Station_Ruhrort/LConn2 -- Stockum_Ost+West_CN_35818134_220000_CN_35818137_220000/RConn2
  T_35818134_220000;110000_Station_Ruhrort/LConn3 -- Stockum_Ost+West_CN_35818134_220000_CN_35818137_220000/RConn3
  T_35818522_220000_/LConn1 -- _CN_35818137_220000_CN_35818522_220000/RConn1
  T_35818522_220000_/LConn2 -- _CN_35818137_220000_CN_35818522_220000/RConn2
  T_35818522_220000_/LConn3 -- _CN_35818137_220000_CN_35818522_220000/RConn3
  _CN_66038431_220000_CN_24667346_220000/RConn1 -- T_66038431_220000;110000_Station_Laer/LConn1 -- _CN_66038431_220000_CN131986820/LConn1 -- _CN_66038431_220000_CN_113546939_220000/RConn1 -- _CN_66038431_220000_CN_28452784_220000/RConn1
  _CN_66038431_220000_CN_24667346_220000/RConn2 -- T_66038431_220000;110000_Station_Laer/LConn2 -- _CN_66038431_220000_CN131986820/LConn2 -- _CN_66038431_220000_CN_113546939_220000/RConn2 -- _CN_66038431_220000_CN_28452784_220000/RConn2
  _CN_66038431_220000_CN_24667346_220000/RConn3 -- T_66038431_220000;110000_Station_Laer/LConn3 -- _CN_66038431_220000_CN131986820/LConn3 -- _CN_66038431_220000_CN_113546939_220000/RConn3 -- _CN_66038431_220000_CN_28452784_220000/RConn3
  G_131986820_Koepchenwerk/RConn1 -- _CN_66038431_220000_CN131986820/RConn1
  G_131986820_Koepchenwerk/RConn2 -- _CN_66038431_220000_CN131986820/RConn2
  G_131986820_Koepchenwerk/RConn3 -- _CN_66038431_220000_CN131986820/RConn3
  T_39688875_220000_Umspannwerk_Windpark_Iven/LConn1 -- 316_CN_39688875_220000_CN_39437430_220000/LConn1
  T_39688875_220000_Umspannwerk_Windpark_Iven/LConn2 -- 316_CN_39688875_220000_CN_39437430_220000/LConn2
  T_39688875_220000_Umspannwerk_Windpark_Iven/LConn3 -- 316_CN_39688875_220000_CN_39437430_220000/LConn3
  316_CN_39688875_220000_CN_39437430_220000/RConn1 -- T_39437430_220000;110000_Pasewalk/LConn1 -- 306_CN_39437430_220000_CN_30039908_220000/LConn1 -- 306_CN_39437430_220000_CN215092049/RConn1 -- 306_CN_39437430_220000_CN_39428980_220000/LConn1
  316_CN_39688875_220000_CN_39437430_220000/RConn2 -- T_39437430_220000;110000_Pasewalk/LConn2 -- 306_CN_39437430_220000_CN_30039908_220000/LConn2 -- 306_CN_39437430_220000_CN215092049/RConn2 -- 306_CN_39437430_220000_CN_39428980_220000/LConn2
  316_CN_39688875_220000_CN_39437430_220000/RConn3 -- T_39437430_220000;110000_Pasewalk/LConn3 -- 306_CN_39437430_220000_CN_30039908_220000/LConn3 -- 306_CN_39437430_220000_CN215092049/RConn3 -- 306_CN_39437430_220000_CN_39428980_220000/LConn3
  _CN_32318130_220000_CN_29389718_220000/LConn1 -- T_32318130_220000;110000_Bentwisch/LConn1 -- _CN_32318130_220000_CN_32062544_220000/RConn1
  _CN_32318130_220000_CN_29389718_220000/LConn2 -- T_32318130_220000;110000_Bentwisch/LConn2 -- _CN_32318130_220000_CN_32062544_220000/RConn2
  _CN_32318130_220000_CN_29389718_220000/LConn3 -- T_32318130_220000;110000_Bentwisch/LConn3 -- _CN_32318130_220000_CN_32062544_220000/RConn3
  _CN_32318130_220000_CN_29389718_220000/RConn1 -- T_29389718_220000;110000_Umspannwerk_Lüdershagen/LConn1 -- 313_CN_29389718_220000_CN_29877599_220000/LConn1
  _CN_32318130_220000_CN_29389718_220000/RConn2 -- T_29389718_220000;110000_Umspannwerk_Lüdershagen/LConn2 -- 313_CN_29389718_220000_CN_29877599_220000/LConn2
  _CN_32318130_220000_CN_29389718_220000/RConn3 -- T_29389718_220000;110000_Umspannwerk_Lüdershagen/LConn3 -- 313_CN_29389718_220000_CN_29877599_220000/LConn3
  Raitersaich___Trennfeld;Trennfeld___Aschaffenburg_CN_24765111_220000_CN_133349218_220000/LConn1 -- T_24765111_220000;110000_Umspannwerk_Trennfeld/LConn1 -- Raitersaich___Trennfeld;Trennfeld___Aschaffenburg_CN_24765111_220000_CN_55069713_220000/LConn1 -- Raitersaich___Trennfeld;Trennfeld___Aschaffenburg_CN_24765111_220000_CN_24705761_220000/RConn1
  Raitersaich___Trennfeld;Trennfeld___Aschaffenburg_CN_24765111_220000_CN_133349218_220000/LConn2 -- T_24765111_220000;110000_Umspannwerk_Trennfeld/LConn2 -- Raitersaich___Trennfeld;Trennfeld___Aschaffenburg_CN_24765111_220000_CN_55069713_220000/LConn2 -- Raitersaich___Trennfeld;Trennfeld___Aschaffenburg_CN_24765111_220000_CN_24705761_220000/RConn2
  Raitersaich___Trennfeld;Trennfeld___Aschaffenburg_CN_24765111_220000_CN_133349218_220000/LConn3 -- T_24765111_220000;110000_Umspannwerk_Trennfeld/LConn3 -- Raitersaich___Trennfeld;Trennfeld___Aschaffenburg_CN_24765111_220000_CN_55069713_220000/LConn3 -- Raitersaich___Trennfeld;Trennfeld___Aschaffenburg_CN_24765111_220000_CN_24705761_220000/RConn3
  Raitersaich___Trennfeld;Trennfeld___Aschaffenburg_CN_24765111_220000_CN_133349218_220000/RConn1 -- T_133349218_220000;110000_Umspannwerk_Ludersheim/LConn1 -- Ludersheim___Schwandorf_CN_133349218_220000_CN_28956649_220000/RConn1 -- LU_SIT_CN_24759324_220000_CN_133349218_220000/LConn1
  Raitersaich___Trennfeld;Trennfeld___Aschaffenburg_CN_24765111_220000_CN_133349218_220000/RConn2 -- T_133349218_220000;110000_Umspannwerk_Ludersheim/LConn2 -- Ludersheim___Schwandorf_CN_133349218_220000_CN_28956649_220000/RConn2 -- LU_SIT_CN_24759324_220000_CN_133349218_220000/LConn2
  Raitersaich___Trennfeld;Trennfeld___Aschaffenburg_CN_24765111_220000_CN_133349218_220000/RConn3 -- T_133349218_220000;110000_Umspannwerk_Ludersheim/LConn3 -- Ludersheim___Schwandorf_CN_133349218_220000_CN_28956649_220000/RConn3 -- LU_SIT_CN_24759324_220000_CN_133349218_220000/LConn3
  Raitersaich___Trennfeld;Trennfeld___Aschaffenburg_CN_24765111_220000_CN_55069713_220000/RConn1 -- T_55069713_380000;220000;110000_Umspannwerk_Aschaffenburg/RConn1 -- 2205;III;IIII_CN_55069713_220000_CN_42411962_220000/LConn1 -- L_55069713/LConn1
  Raitersaich___Trennfeld;Trennfeld___Aschaffenburg_CN_24765111_220000_CN_55069713_220000/RConn2 -- T_55069713_380000;220000;110000_Umspannwerk_Aschaffenburg/RConn2 -- 2205;III;IIII_CN_55069713_220000_CN_42411962_220000/LConn2 -- L_55069713/LConn2
  Raitersaich___Trennfeld;Trennfeld___Aschaffenburg_CN_24765111_220000_CN_55069713_220000/RConn3 -- T_55069713_380000;220000;110000_Umspannwerk_Aschaffenburg/RConn3 -- 2205;III;IIII_CN_55069713_220000_CN_42411962_220000/LConn3 -- L_55069713/LConn3
  T_109917397_380000_Freiberg_Nord_(380_kV)/LConn1 -- Schmölln___Dresden_Süd___Röhrsdorf_CN_157807291_380000_CN_109917397_380000/RConn1
  T_109917397_380000_Freiberg_Nord_(380_kV)/LConn2 -- Schmölln___Dresden_Süd___Röhrsdorf_CN_157807291_380000_CN_109917397_380000/RConn2
  T_109917397_380000_Freiberg_Nord_(380_kV)/LConn3 -- Schmölln___Dresden_Süd___Röhrsdorf_CN_157807291_380000_CN_109917397_380000/RConn3
  T_23241863_380000;110000_Umspannwerk_DD_Süd/LConn1 -- Schmölln___Dresden_Süd___Röhrsdorf_CN_157807291_380000_CN_23241863_380000/RConn1
  T_23241863_380000;110000_Umspannwerk_DD_Süd/LConn2 -- Schmölln___Dresden_Süd___Röhrsdorf_CN_157807291_380000_CN_23241863_380000/RConn2
  T_23241863_380000;110000_Umspannwerk_DD_Süd/LConn3 -- Schmölln___Dresden_Süd___Röhrsdorf_CN_157807291_380000_CN_23241863_380000/RConn3
  Leitung_3018_CN_24604789_380000_CN_24230738_380000/RConn1 -- T_24230738_380000;110000_Eickum/LConn1 -- _CN_24230738_380000_CN_24264701_380000/LConn1
  Leitung_3018_CN_24604789_380000_CN_24230738_380000/RConn2 -- T_24230738_380000;110000_Eickum/LConn2 -- _CN_24230738_380000_CN_24264701_380000/LConn2
  Leitung_3018_CN_24604789_380000_CN_24230738_380000/RConn3 -- T_24230738_380000;110000_Eickum/LConn3 -- _CN_24230738_380000_CN_24264701_380000/LConn3
  _CN_26383042_380000_CN_24264701_380000/RConn1 -- T_24264701_380000;220000;110000_Umspannwerk_Bechterdissen/LConn1 -- _CN_24230738_380000_CN_24264701_380000/RConn1 -- _CN_25943440_380000_CN_24264701_380000/RConn1
  _CN_26383042_380000_CN_24264701_380000/RConn2 -- T_24264701_380000;220000;110000_Umspannwerk_Bechterdissen/LConn2 -- _CN_24230738_380000_CN_24264701_380000/RConn2 -- _CN_25943440_380000_CN_24264701_380000/RConn2
  _CN_26383042_380000_CN_24264701_380000/RConn3 -- T_24264701_380000;220000;110000_Umspannwerk_Bechterdissen/LConn3 -- _CN_24230738_380000_CN_24264701_380000/RConn3 -- _CN_25943440_380000_CN_24264701_380000/RConn3
  _CN_26383042_220000_CN_26611458_220000/RConn1 -- T_26383042_380000;220000;110000;10000_Umspannwerk_Blankenhagen/RConn1 -- _CN_26383042_220000_CN_37764852_220000/RConn1 -- _CN_26383042_220000_CN_39229429_220000/LConn1 -- L_26383042/LConn1
  _CN_26383042_220000_CN_26611458_220000/RConn2 -- T_26383042_380000;220000;110000;10000_Umspannwerk_Blankenhagen/RConn2 -- _CN_26383042_220000_CN_37764852_220000/RConn2 -- _CN_26383042_220000_CN_39229429_220000/LConn2 -- L_26383042/LConn2
  _CN_26383042_220000_CN_26611458_220000/RConn3 -- T_26383042_380000;220000;110000;10000_Umspannwerk_Blankenhagen/RConn3 -- _CN_26383042_220000_CN_37764852_220000/RConn3 -- _CN_26383042_220000_CN_39229429_220000/LConn3 -- L_26383042/LConn3
  T_39229429_220000;110000_Station_Hesseln/LConn1 -- _CN_26383042_220000_CN_39229429_220000/RConn1
  T_39229429_220000;110000_Station_Hesseln/LConn2 -- _CN_26383042_220000_CN_39229429_220000/RConn2
  T_39229429_220000;110000_Station_Hesseln/LConn3 -- _CN_26383042_220000_CN_39229429_220000/RConn3
  306_CN_39437430_220000_CN_30039908_220000/RConn1 -- T_30039908_380000;220000_Bertikow/RConn1 -- L_30039908/LConn1
  306_CN_39437430_220000_CN_30039908_220000/RConn2 -- T_30039908_380000;220000_Bertikow/RConn2 -- L_30039908/LConn2
  306_CN_39437430_220000_CN_30039908_220000/RConn3 -- T_30039908_380000;220000_Bertikow/RConn3 -- L_30039908/LConn3
  T_39428980_220000;110000_Vierraden/LConn1 -- 306_CN_39437430_220000_CN_39428980_220000/RConn1
  T_39428980_220000;110000_Vierraden/LConn2 -- 306_CN_39437430_220000_CN_39428980_220000/RConn2
  T_39428980_220000;110000_Vierraden/LConn3 -- 306_CN_39437430_220000_CN_39428980_220000/RConn3
  T_90109304_220000_UA_Dillinger_Hütte_Mitte/LConn1 -- _CN_82310607_220000_CN_90109304_220000/RConn1
  T_90109304_220000_UA_Dillinger_Hütte_Mitte/LConn2 -- _CN_82310607_220000_CN_90109304_220000/RConn2
  T_90109304_220000_UA_Dillinger_Hütte_Mitte/LConn3 -- _CN_82310607_220000_CN_90109304_220000/RConn3
  Irsching___Raitersaich_CN_24705761_380000_CN_24768051_380000/RConn1 -- T_24768051_380000;220000;110000_Ingolstadt/LConn1 -- Irsching___Raitersaich_CN_137602559_380000_CN_24768051_380000/LConn1
  Irsching___Raitersaich_CN_24705761_380000_CN_24768051_380000/RConn2 -- T_24768051_380000;220000;110000_Ingolstadt/LConn2 -- Irsching___Raitersaich_CN_137602559_380000_CN_24768051_380000/LConn2
  Irsching___Raitersaich_CN_24705761_380000_CN_24768051_380000/RConn3 -- T_24768051_380000;220000;110000_Ingolstadt/LConn3 -- Irsching___Raitersaich_CN_137602559_380000_CN_24768051_380000/LConn3
  Tiengen___Stockach_CN_31367936_220000_CN_102743264_220000/LConn1 -- T_31367936_220000;110000_Umspannwerk_Stockach/LConn1 -- Tiengen___Stockach_CN_31367936_220000_CN_31367937_220000/LConn1
  Tiengen___Stockach_CN_31367936_220000_CN_102743264_220000/LConn2 -- T_31367936_220000;110000_Umspannwerk_Stockach/LConn2 -- Tiengen___Stockach_CN_31367936_220000_CN_31367937_220000/LConn2
  Tiengen___Stockach_CN_31367936_220000_CN_102743264_220000/LConn3 -- T_31367936_220000;110000_Umspannwerk_Stockach/LConn3 -- Tiengen___Stockach_CN_31367936_220000_CN_31367937_220000/LConn3
  T_102743264_220000;110000_Beuren/LConn1 -- Tiengen___Stockach_CN_31367936_220000_CN_102743264_220000/RConn1
  T_102743264_220000;110000_Beuren/LConn2 -- Tiengen___Stockach_CN_31367936_220000_CN_102743264_220000/RConn2
  T_102743264_220000;110000_Beuren/LConn3 -- Tiengen___Stockach_CN_31367936_220000_CN_102743264_220000/RConn3
  Tiengen___Stockach_CN_31367936_220000_CN_31367937_220000/RConn1 -- T_31367937_220000;110000_Umspannwerk_Gurtweil/LConn1 -- Tiengen___Schlücht_1x_220_kV_CN_31367937_220000_CN_31367940_220000/LConn1 -- _CN_31367937_220000_CN_87653464_220000/RConn1
  Tiengen___Stockach_CN_31367936_220000_CN_31367937_220000/RConn2 -- T_31367937_220000;110000_Umspannwerk_Gurtweil/LConn2 -- Tiengen___Schlücht_1x_220_kV_CN_31367937_220000_CN_31367940_220000/LConn2 -- _CN_31367937_220000_CN_87653464_220000/RConn2
  Tiengen___Stockach_CN_31367936_220000_CN_31367937_220000/RConn3 -- T_31367937_220000;110000_Umspannwerk_Gurtweil/LConn3 -- Tiengen___Schlücht_1x_220_kV_CN_31367937_220000_CN_31367940_220000/LConn3 -- _CN_31367937_220000_CN_87653464_220000/RConn3
  Tiengen___Schlücht_1x_220_kV_CN_31367937_220000_CN_31367940_220000/RConn1 -- T_31367940_380000;220000;110000_Tiengen/RConn1 -- L_31367940/LConn1
  Tiengen___Schlücht_1x_220_kV_CN_31367937_220000_CN_31367940_220000/RConn2 -- T_31367940_380000;220000;110000_Tiengen/RConn2 -- L_31367940/LConn2
  Tiengen___Schlücht_1x_220_kV_CN_31367937_220000_CN_31367940_220000/RConn3 -- T_31367940_380000;220000;110000_Tiengen/RConn3 -- L_31367940/LConn3
  _CN_77697810_380000_CN23802422/RConn1 -- T_77697810_380000_Isar/LConn1 -- _CN_77697810_380000_CN_24976300_380000/LConn1
  _CN_77697810_380000_CN23802422/RConn2 -- T_77697810_380000_Isar/LConn2 -- _CN_77697810_380000_CN_24976300_380000/LConn2
  _CN_77697810_380000_CN23802422/RConn3 -- T_77697810_380000_Isar/LConn3 -- _CN_77697810_380000_CN_24976300_380000/LConn3
  T_24976300_380000;220000;110000_Umspannwerk_Pleinting/LConn1 -- _CN_77697810_380000_CN_24976300_380000/RConn1
  T_24976300_380000;220000;110000_Umspannwerk_Pleinting/LConn2 -- _CN_77697810_380000_CN_24976300_380000/RConn2
  T_24976300_380000;220000;110000_Umspannwerk_Pleinting/LConn3 -- _CN_77697810_380000_CN_24976300_380000/RConn3
  G_152261126_Rheinhafen_Dampfkraftwerk/RConn1 -- 7563_CN_272646943_380000_CN152261126/RConn1
  G_152261126_Rheinhafen_Dampfkraftwerk/RConn2 -- 7563_CN_272646943_380000_CN152261126/RConn2
  G_152261126_Rheinhafen_Dampfkraftwerk/RConn3 -- 7563_CN_272646943_380000_CN152261126/RConn3
  T_147878692_380000;110000_Umrichterwerk_Neckarwestheim/LConn1 -- _CN_147878692_380000_CN23547196/RConn1
  T_147878692_380000;110000_Umrichterwerk_Neckarwestheim/LConn2 -- _CN_147878692_380000_CN23547196/RConn2
  T_147878692_380000;110000_Umrichterwerk_Neckarwestheim/LConn3 -- _CN_147878692_380000_CN23547196/RConn3
  T_118928165_220000_Benteler_Stahlwerk/LConn1 -- 220kV_Benteler_CN_118928165_220000_CN_61918154_220000/RConn1
  T_118928165_220000_Benteler_Stahlwerk/LConn2 -- 220kV_Benteler_CN_118928165_220000_CN_61918154_220000/RConn2
  T_118928165_220000_Benteler_Stahlwerk/LConn3 -- 220kV_Benteler_CN_118928165_220000_CN_61918154_220000/RConn3
  T_90807341_220000;110000_Umspannwerk_Kempten_Au/LConn1 -- _CN_46766896_220000_CN_90807341_220000/RConn1
  T_90807341_220000;110000_Umspannwerk_Kempten_Au/LConn2 -- _CN_46766896_220000_CN_90807341_220000/RConn2
  T_90807341_220000;110000_Umspannwerk_Kempten_Au/LConn3 -- _CN_46766896_220000_CN_90807341_220000/RConn3
  T_23907283_380000;110000_Hauptumspannwerk_Menzing/LConn1 -- OBA___MZ_CN_18629425_380000_CN_23907283_380000/RConn1
  T_23907283_380000;110000_Hauptumspannwerk_Menzing/LConn2 -- OBA___MZ_CN_18629425_380000_CN_23907283_380000/RConn2
  T_23907283_380000;110000_Hauptumspannwerk_Menzing/LConn3 -- OBA___MZ_CN_18629425_380000_CN_23907283_380000/RConn3
  T_111973179_220000;110000_Station_Münster/LConn1 -- _CN_111973179_220000_CN_42861703_220000/RConn1
  T_111973179_220000;110000_Station_Münster/LConn2 -- _CN_111973179_220000_CN_42861703_220000/RConn2
  T_111973179_220000;110000_Station_Münster/LConn3 -- _CN_111973179_220000_CN_42861703_220000/RConn3
  3021_UW_Lüneburg___UW_Stadorf_CN_28343121_380000_CN_28327356_380000/RConn1 -- T_28327356_380000;110000_Lüneburg/LConn1 -- _CN_23366603_380000_CN_28327356_380000/RConn1
  3021_UW_Lüneburg___UW_Stadorf_CN_28343121_380000_CN_28327356_380000/RConn2 -- T_28327356_380000;110000_Lüneburg/LConn2 -- _CN_23366603_380000_CN_28327356_380000/RConn2
  3021_UW_Lüneburg___UW_Stadorf_CN_28343121_380000_CN_28327356_380000/RConn3 -- T_28327356_380000;110000_Lüneburg/LConn3 -- _CN_23366603_380000_CN_28327356_380000/RConn3
  _CN_29309786_380000_CN_156673636_380000/RConn1 -- T_156673636_380000;110000_Umspannwerk_Borken/LConn1 -- Leitung_3212;Leitung_3213_CN_156673636_380000_CN_41072584_380000/LConn1 -- _CN_202747445_380000_CN_156673636_380000/LConn1 -- _CN_156673636_380000_CN_156960655_380000/LConn1 -- Leitung_3212;Leitung_3213_CN_156673636_380000_CN_41232144_380000/RConn1
  _CN_29309786_380000_CN_156673636_380000/RConn2 -- T_156673636_380000;110000_Umspannwerk_Borken/LConn2 -- Leitung_3212;Leitung_3213_CN_156673636_380000_CN_41072584_380000/LConn2 -- _CN_202747445_380000_CN_156673636_380000/LConn2 -- _CN_156673636_380000_CN_156960655_380000/LConn2 -- Leitung_3212;Leitung_3213_CN_156673636_380000_CN_41232144_380000/RConn2
  _CN_29309786_380000_CN_156673636_380000/RConn3 -- T_156673636_380000;110000_Umspannwerk_Borken/LConn3 -- Leitung_3212;Leitung_3213_CN_156673636_380000_CN_41072584_380000/LConn3 -- _CN_202747445_380000_CN_156673636_380000/LConn3 -- _CN_156673636_380000_CN_156960655_380000/LConn3 -- Leitung_3212;Leitung_3213_CN_156673636_380000_CN_41232144_380000/RConn3
  _CN_29309786_380000_CN_148446247_380000/RConn1 -- T_148446247_380000;110000_UW_Dipperz/LConn1 -- AS_GKRO;GKRO_GR_I;DIP_GKB_I;_II_CN_42410916_380000_CN_148446247_380000/RConn1
  _CN_29309786_380000_CN_148446247_380000/RConn2 -- T_148446247_380000;110000_UW_Dipperz/LConn2 -- AS_GKRO;GKRO_GR_I;DIP_GKB_I;_II_CN_42410916_380000_CN_148446247_380000/RConn2
  _CN_29309786_380000_CN_148446247_380000/RConn3 -- T_148446247_380000;110000_UW_Dipperz/LConn3 -- AS_GKRO;GKRO_GR_I;DIP_GKB_I;_II_CN_42410916_380000_CN_148446247_380000/RConn3
  T_232833796_220000_/LConn1 -- _CN_232833796_220000_CN_133342285_220000/RConn1
  T_232833796_220000_/LConn2 -- _CN_232833796_220000_CN_133342285_220000/RConn2
  T_232833796_220000_/LConn3 -- _CN_232833796_220000_CN_133342285_220000/RConn3
  Leitung_2014_CN_43072656_220000_CN_29103809_220000/RConn1 -- T_29103809_220000;110000_Umspannwerk_Rosdorf/LConn1 -- Leitung_2013_CN_172997498_220000_CN_29103809_220000/LConn1
  Leitung_2014_CN_43072656_220000_CN_29103809_220000/RConn2 -- T_29103809_220000;110000_Umspannwerk_Rosdorf/LConn2 -- Leitung_2013_CN_172997498_220000_CN_29103809_220000/LConn2
  Leitung_2014_CN_43072656_220000_CN_29103809_220000/RConn3 -- T_29103809_220000;110000_Umspannwerk_Rosdorf/LConn3 -- Leitung_2013_CN_172997498_220000_CN_29103809_220000/LConn3
  T_254326606_380000;110000_Umspannwerk_Bruchsal_Kändelweg/LConn1 -- Philippsburg___Pulverdingen_CN_43688805_380000_CN_254326606_380000/RConn1
  T_254326606_380000;110000_Umspannwerk_Bruchsal_Kändelweg/LConn2 -- Philippsburg___Pulverdingen_CN_43688805_380000_CN_254326606_380000/RConn2
  T_254326606_380000;110000_Umspannwerk_Bruchsal_Kändelweg/LConn3 -- Philippsburg___Pulverdingen_CN_43688805_380000_CN_254326606_380000/RConn3
  _CN_89176939_220000_CN_151967290_220000/RConn1 -- T_89176939_220000_SA_Bauler/LConn1 -- _CN_89176939_220000_CN_89176956_220000/LConn1
  _CN_89176939_220000_CN_151967290_220000/RConn2 -- T_89176939_220000_SA_Bauler/LConn2 -- _CN_89176939_220000_CN_89176956_220000/LConn2
  _CN_89176939_220000_CN_151967290_220000/RConn3 -- T_89176939_220000_SA_Bauler/LConn3 -- _CN_89176939_220000_CN_89176956_220000/LConn3
  T_89176956_220000_Vianden/LConn1 -- _CN_89176939_220000_CN_89176956_220000/RConn1
  T_89176956_220000_Vianden/LConn2 -- _CN_89176939_220000_CN_89176956_220000/RConn2
  T_89176956_220000_Vianden/LConn3 -- _CN_89176939_220000_CN_89176956_220000/RConn3
  _CN_24042358_380000_CN_42410916_380000/RConn1 -- T_24042358_380000;110000_Umspannwerk_Karben/LConn1 -- _CN_24042358_380000_CN_202747445_380000/LConn1 -- _CN_24042358_380000_CN_62061952_380000/LConn1
  _CN_24042358_380000_CN_42410916_380000/RConn2 -- T_24042358_380000;110000_Umspannwerk_Karben/LConn2 -- _CN_24042358_380000_CN_202747445_380000/LConn2 -- _CN_24042358_380000_CN_62061952_380000/LConn2
  _CN_24042358_380000_CN_42410916_380000/RConn3 -- T_24042358_380000;110000_Umspannwerk_Karben/LConn3 -- _CN_24042358_380000_CN_202747445_380000/LConn3 -- _CN_24042358_380000_CN_62061952_380000/LConn3
  _CN_24042358_380000_CN_202747445_380000/RConn1 -- T_202747445_380000;110000_Umspannwerk_Gießen_Nord/LConn1 -- _CN_24536211_380000_CN_202747445_380000/LConn1 -- _CN_202747445_380000_CN_156673636_380000/RConn1
  _CN_24042358_380000_CN_202747445_380000/RConn2 -- T_202747445_380000;110000_Umspannwerk_Gießen_Nord/LConn2 -- _CN_24536211_380000_CN_202747445_380000/LConn2 -- _CN_202747445_380000_CN_156673636_380000/RConn2
  _CN_24042358_380000_CN_202747445_380000/RConn3 -- T_202747445_380000;110000_Umspannwerk_Gießen_Nord/LConn3 -- _CN_24536211_380000_CN_202747445_380000/LConn3 -- _CN_202747445_380000_CN_156673636_380000/RConn3
  T_62061952_380000_Umspannwerk_Frankfurt_Südwest/LConn1 -- _CN_24042358_380000_CN_62061952_380000/RConn1
  T_62061952_380000_Umspannwerk_Frankfurt_Südwest/LConn2 -- _CN_24042358_380000_CN_62061952_380000/RConn2
  T_62061952_380000_Umspannwerk_Frankfurt_Südwest/LConn3 -- _CN_24042358_380000_CN_62061952_380000/RConn3
  Leitung_2013_CN_172997498_220000_CN_29103809_220000/RConn1 -- T_172997498_220000;110000_Sandershausen/LConn1 -- _CN_172997498_220000_CN_274630377_220000/LConn1
  Leitung_2013_CN_172997498_220000_CN_29103809_220000/RConn2 -- T_172997498_220000;110000_Sandershausen/LConn2 -- _CN_172997498_220000_CN_274630377_220000/LConn2
  Leitung_2013_CN_172997498_220000_CN_29103809_220000/RConn3 -- T_172997498_220000;110000_Sandershausen/LConn3 -- _CN_172997498_220000_CN_274630377_220000/LConn3
  _CN_172997498_220000_CN_274630377_220000/RConn1 -- T_274630377_380000;220000;110000_Umspannanlage_Würgassen/RConn1 -- L_274630377/LConn1
  _CN_172997498_220000_CN_274630377_220000/RConn2 -- T_274630377_380000;220000;110000_Umspannanlage_Würgassen/RConn2 -- L_274630377/LConn2
  _CN_172997498_220000_CN_274630377_220000/RConn3 -- T_274630377_380000;220000;110000_Umspannanlage_Würgassen/RConn3 -- L_274630377/LConn3
  207_CN_27124619_220000_CN_33148774_220000/LConn1 -- T_27124619_220000;110000_Kiel_Süd/LConn1 -- 207_CN_27124619_220000_CN_27646106_220000/LConn1 -- _CN_27124619_220000_CN149869150/LConn1
  207_CN_27124619_220000_CN_33148774_220000/LConn2 -- T_27124619_220000;110000_Kiel_Süd/LConn2 -- 207_CN_27124619_220000_CN_27646106_220000/LConn2 -- _CN_27124619_220000_CN149869150/LConn2
  207_CN_27124619_220000_CN_33148774_220000/LConn3 -- T_27124619_220000;110000_Kiel_Süd/LConn3 -- 207_CN_27124619_220000_CN_27646106_220000/LConn3 -- _CN_27124619_220000_CN149869150/LConn3
  207_CN_27124619_220000_CN_33148774_220000/RConn1 -- T_33148774_220000;110000_Audorf/LConn1 -- _CN_87952821_220000_CN_33148774_220000/LConn1 -- _CN_28008024_220000_CN_33148774_220000/RConn1
  207_CN_27124619_220000_CN_33148774_220000/RConn2 -- T_33148774_220000;110000_Audorf/LConn2 -- _CN_87952821_220000_CN_33148774_220000/LConn2 -- _CN_28008024_220000_CN_33148774_220000/RConn2
  207_CN_27124619_220000_CN_33148774_220000/RConn3 -- T_33148774_220000;110000_Audorf/LConn3 -- _CN_87952821_220000_CN_33148774_220000/LConn3 -- _CN_28008024_220000_CN_33148774_220000/RConn3
  T_27646106_220000;110000_Umspannwerk_Kiel_West/LConn1 -- 207_CN_27124619_220000_CN_27646106_220000/RConn1
  T_27646106_220000;110000_Umspannwerk_Kiel_West/LConn2 -- 207_CN_27124619_220000_CN_27646106_220000/RConn2
  T_27646106_220000;110000_Umspannwerk_Kiel_West/LConn3 -- 207_CN_27124619_220000_CN_27646106_220000/RConn3
  G_149869150_Gemeinschaftskraftwerk_Kiel/RConn1 -- _CN_27124619_220000_CN149869150/RConn1
  G_149869150_Gemeinschaftskraftwerk_Kiel/RConn2 -- _CN_27124619_220000_CN149869150/RConn2
  G_149869150_Gemeinschaftskraftwerk_Kiel/RConn3 -- _CN_27124619_220000_CN149869150/RConn3
  T_59925390_380000;110000_Station_Karnap/LConn1 -- _CN_59925390_380000_CN_113546939_380000/RConn1
  T_59925390_380000;110000_Station_Karnap/LConn2 -- _CN_59925390_380000_CN_113546939_380000/RConn2
  T_59925390_380000;110000_Station_Karnap/LConn3 -- _CN_59925390_380000_CN_113546939_380000/RConn3
  _CN_30622610_220000_CN55015415/LConn1 -- T_30622610_380000;220000;110000_Umspannwerk_Kernkraftwerk_Brunsbüttel/RConn1 -- L_30622610/LConn1
  _CN_30622610_220000_CN55015415/LConn2 -- T_30622610_380000;220000;110000_Umspannwerk_Kernkraftwerk_Brunsbüttel/RConn2 -- L_30622610/LConn2
  _CN_30622610_220000_CN55015415/LConn3 -- T_30622610_380000;220000;110000_Umspannwerk_Kernkraftwerk_Brunsbüttel/RConn3 -- L_30622610/LConn3
  _CN_30622610_220000_CN55015415/RConn1 -- G_55015415_Gasturbinenkraftwerk_Itzehoe/RConn1 -- _CN_60032354_220000_CN55015415/LConn1
  _CN_30622610_220000_CN55015415/RConn2 -- G_55015415_Gasturbinenkraftwerk_Itzehoe/RConn2 -- _CN_60032354_220000_CN55015415/LConn2
  _CN_30622610_220000_CN55015415/RConn3 -- G_55015415_Gasturbinenkraftwerk_Itzehoe/RConn3 -- _CN_60032354_220000_CN55015415/LConn3
  313_CN_29389718_220000_CN_29877599_220000/RConn1 -- T_29877599_380000;220000_Umspannwerk_Lubmin/RConn1 -- L_29877599/LConn1
  313_CN_29389718_220000_CN_29877599_220000/RConn2 -- T_29877599_380000;220000_Umspannwerk_Lubmin/RConn2 -- L_29877599/LConn2
  313_CN_29389718_220000_CN_29877599_220000/RConn3 -- T_29877599_380000;220000_Umspannwerk_Lubmin/RConn3 -- L_29877599/LConn3
  T_31019937_380000;220000;110000_Vöhringen_LEW/LConn1 -- _CN_31019937_380000_CN_85523877_380000/RConn1
  T_31019937_380000;220000;110000_Vöhringen_LEW/LConn2 -- _CN_31019937_380000_CN_85523877_380000/RConn2
  T_31019937_380000;220000;110000_Vöhringen_LEW/LConn3 -- _CN_31019937_380000_CN_85523877_380000/RConn3
  Iller_Ltg__CN_31019937_220000_CN_41389594_220000/RConn1 -- T_41389594_380000;220000;110000_Umspannwerk_Dellmensingen/RConn1 -- Dellmensingen___Obermooweiler;Dellmensingen_Ost_CN_41389594_220000_CN_25306752_220000/RConn1 -- L_41389594/LConn1
  Iller_Ltg__CN_31019937_220000_CN_41389594_220000/RConn2 -- T_41389594_380000;220000;110000_Umspannwerk_Dellmensingen/RConn2 -- Dellmensingen___Obermooweiler;Dellmensingen_Ost_CN_41389594_220000_CN_25306752_220000/RConn2 -- L_41389594/LConn2
  Iller_Ltg__CN_31019937_220000_CN_41389594_220000/RConn3 -- T_41389594_380000;220000;110000_Umspannwerk_Dellmensingen/RConn3 -- Dellmensingen___Obermooweiler;Dellmensingen_Ost_CN_41389594_220000_CN_25306752_220000/RConn3 -- L_41389594/LConn3
  _CN_42410916_220000_CN_42411962_220000/LConn1 -- T_42410916_380000;220000_Umspannwerk_Großkrotzenburg/RConn1 -- _CN_42410916_220000_CN145861680/LConn1 -- L_42410916/LConn1
  _CN_42410916_220000_CN_42411962_220000/LConn2 -- T_42410916_380000;220000_Umspannwerk_Großkrotzenburg/RConn2 -- _CN_42410916_220000_CN145861680/LConn2 -- L_42410916/LConn2
  _CN_42410916_220000_CN_42411962_220000/LConn3 -- T_42410916_380000;220000_Umspannwerk_Großkrotzenburg/RConn3 -- _CN_42410916_220000_CN145861680/LConn3 -- L_42410916/LConn3
  _CN_42410916_220000_CN_42411962_220000/RConn1 -- T_42411962_220000;110000_Kraftwerkseinspeisung_Staudinger/LConn1 -- _CN_23881272_220000_CN_42411962_220000/LConn1 -- _CN_42411962_220000_CN145861680/LConn1 -- 2205;III;IIII_CN_55069713_220000_CN_42411962_220000/RConn1
  _CN_42410916_220000_CN_42411962_220000/RConn2 -- T_42411962_220000;110000_Kraftwerkseinspeisung_Staudinger/LConn2 -- _CN_23881272_220000_CN_42411962_220000/LConn2 -- _CN_42411962_220000_CN145861680/LConn2 -- 2205;III;IIII_CN_55069713_220000_CN_42411962_220000/RConn2
  _CN_42410916_220000_CN_42411962_220000/RConn3 -- T_42411962_220000;110000_Kraftwerkseinspeisung_Staudinger/LConn3 -- _CN_23881272_220000_CN_42411962_220000/LConn3 -- _CN_42411962_220000_CN145861680/LConn3 -- 2205;III;IIII_CN_55069713_220000_CN_42411962_220000/RConn3
  _CN_42410916_220000_CN145861680/RConn1 -- G_145861680_Kraftwerk_Staudinger/RConn1 -- _CN_42411962_220000_CN145861680/RConn1
  _CN_42410916_220000_CN145861680/RConn2 -- G_145861680_Kraftwerk_Staudinger/RConn2 -- _CN_42411962_220000_CN145861680/RConn2
  _CN_42410916_220000_CN145861680/RConn3 -- G_145861680_Kraftwerk_Staudinger/RConn3 -- _CN_42411962_220000_CN145861680/RConn3
  T_55069713_380000;220000;110000_Umspannwerk_Aschaffenburg/LConn1 -- AS_GKRO;GKRO_GR_I;DIP_GKB_I;_II_CN_42410916_380000_CN_55069713_380000/RConn1
  T_55069713_380000;220000;110000_Umspannwerk_Aschaffenburg/LConn2 -- AS_GKRO;GKRO_GR_I;DIP_GKB_I;_II_CN_42410916_380000_CN_55069713_380000/RConn2
  T_55069713_380000;220000;110000_Umspannwerk_Aschaffenburg/LConn3 -- AS_GKRO;GKRO_GR_I;DIP_GKB_I;_II_CN_42410916_380000_CN_55069713_380000/RConn3
  T_173112252_220000;110000_Crossen/LConn1 -- 212_Röhrsdorf___Crossen_CN_173112252_220000_CN_23117075_220000/RConn1
  T_173112252_220000;110000_Crossen/LConn2 -- 212_Röhrsdorf___Crossen_CN_173112252_220000_CN_23117075_220000/RConn2
  T_173112252_220000;110000_Crossen/LConn3 -- 212_Röhrsdorf___Crossen_CN_173112252_220000_CN_23117075_220000/RConn3
  Conneforde_220_kV_CN_23837631_220000_CN_173178563_220000/RConn1 -- T_23837631_380000;220000;110000_Conneforde/RConn1 -- L_23837631/LConn1
  Conneforde_220_kV_CN_23837631_220000_CN_173178563_220000/RConn2 -- T_23837631_380000;220000;110000_Conneforde/RConn2 -- L_23837631/LConn2
  Conneforde_220_kV_CN_23837631_220000_CN_173178563_220000/RConn3 -- T_23837631_380000;220000;110000_Conneforde/RConn3 -- L_23837631/LConn3
  302_CN_23837631_380000_CN_32076853_380000/RConn1 -- T_32076853_380000;220000;110000_Unterweser/LConn1 -- _CN_32076853_380000_CN_109582315_380000/LConn1 -- 303_CN_44717036_380000_CN_32076853_380000/LConn1
  302_CN_23837631_380000_CN_32076853_380000/RConn2 -- T_32076853_380000;220000;110000_Unterweser/LConn2 -- _CN_32076853_380000_CN_109582315_380000/LConn2 -- 303_CN_44717036_380000_CN_32076853_380000/LConn2
  302_CN_23837631_380000_CN_32076853_380000/RConn3 -- T_32076853_380000;220000;110000_Unterweser/LConn3 -- _CN_32076853_380000_CN_109582315_380000/LConn3 -- 303_CN_44717036_380000_CN_32076853_380000/LConn3
  T_32725958_220000;110000_Karlsruhe_Rintheim/LConn1 -- _CN_32725957_220000_CN_32725958_220000/RConn1
  T_32725958_220000;110000_Karlsruhe_Rintheim/LConn2 -- _CN_32725957_220000_CN_32725958_220000/RConn2
  T_32725958_220000;110000_Karlsruhe_Rintheim/LConn3 -- _CN_32725957_220000_CN_32725958_220000/RConn3
  G_43912398_Kernkraftwerk_Emsland/RConn1 -- 380_kV_Kernkraftwerk_Emsland_CN_61918154_380000_CN43912398/RConn1
  G_43912398_Kernkraftwerk_Emsland/RConn2 -- 380_kV_Kernkraftwerk_Emsland_CN_61918154_380000_CN43912398/RConn2
  G_43912398_Kernkraftwerk_Emsland/RConn3 -- 380_kV_Kernkraftwerk_Emsland_CN_61918154_380000_CN43912398/RConn3
  _CN_61918154_380000_CN49339874/RConn1 -- G_49339874_Erdgaskraftwerk_Emsland/RConn1 -- Emsland_D1|D2|D0_CN_157449983_380000_CN49339874/LConn1
  _CN_61918154_380000_CN49339874/RConn2 -- G_49339874_Erdgaskraftwerk_Emsland/RConn2 -- Emsland_D1|D2|D0_CN_157449983_380000_CN49339874/LConn2
  _CN_61918154_380000_CN49339874/RConn3 -- G_49339874_Erdgaskraftwerk_Emsland/RConn3 -- Emsland_D1|D2|D0_CN_157449983_380000_CN49339874/LConn3
  T_23682013_220000;110000_Hannover_West/LConn1 -- 2016_CN_23682013_220000_CN-2022229/RConn1
  T_23682013_220000;110000_Hannover_West/LConn2 -- 2016_CN_23682013_220000_CN-2022229/RConn2
  T_23682013_220000;110000_Hannover_West/LConn3 -- 2016_CN_23682013_220000_CN-2022229/RConn3
  Maade_schwarz_CN_26455019_220000_CN_23744346_220000/LConn1 -- T_26455019_220000;110000_Voslapp/LConn1 -- 211_CN_26455019_220000_CN_29420322_220000/LConn1
  Maade_schwarz_CN_26455019_220000_CN_23744346_220000/LConn2 -- T_26455019_220000;110000_Voslapp/LConn2 -- 211_CN_26455019_220000_CN_29420322_220000/LConn2
  Maade_schwarz_CN_26455019_220000_CN_23744346_220000/LConn3 -- T_26455019_220000;110000_Voslapp/LConn3 -- 211_CN_26455019_220000_CN_29420322_220000/LConn3
  Maade_schwarz_CN_26455019_220000_CN_23744346_220000/RConn1 -- T_23744346_380000;220000_Umspannwerk_Maade/RConn1 -- 300_CN_23744346_220000_CN26470129/LConn1 -- L_23744346/LConn1 -- 204_CN_173178563_220000_CN_23744346_220000/RConn1 -- Maade_gelb_CN_157421330_220000_CN_23744346_220000/LConn1
  Maade_schwarz_CN_26455019_220000_CN_23744346_220000/RConn2 -- T_23744346_380000;220000_Umspannwerk_Maade/RConn2 -- 300_CN_23744346_220000_CN26470129/LConn2 -- L_23744346/LConn2 -- 204_CN_173178563_220000_CN_23744346_220000/RConn2 -- Maade_gelb_CN_157421330_220000_CN_23744346_220000/LConn2
  Maade_schwarz_CN_26455019_220000_CN_23744346_220000/RConn3 -- T_23744346_380000;220000_Umspannwerk_Maade/RConn3 -- 300_CN_23744346_220000_CN26470129/LConn3 -- L_23744346/LConn3 -- 204_CN_173178563_220000_CN_23744346_220000/RConn3 -- Maade_gelb_CN_157421330_220000_CN_23744346_220000/LConn3
  T_29420322_220000;155000_Inhausen/LConn1 -- 211_CN_26455019_220000_CN_29420322_220000/RConn1
  T_29420322_220000;155000_Inhausen/LConn2 -- 211_CN_26455019_220000_CN_29420322_220000/RConn2
  T_29420322_220000;155000_Inhausen/LConn3 -- 211_CN_26455019_220000_CN_29420322_220000/RConn3
  303_CN_44717036_380000_CN_24493551_380000/LConn1 -- T_44717036_380000;110000_Niedervieland/LConn1 -- 303_CN_44717036_380000_CN_32076853_380000/RConn1 -- 303_CN_44717036_380000_CN313937042/RConn1
  303_CN_44717036_380000_CN_24493551_380000/LConn2 -- T_44717036_380000;110000_Niedervieland/LConn2 -- 303_CN_44717036_380000_CN_32076853_380000/RConn2 -- 303_CN_44717036_380000_CN313937042/RConn2
  303_CN_44717036_380000_CN_24493551_380000/LConn3 -- T_44717036_380000;110000_Niedervieland/LConn3 -- 303_CN_44717036_380000_CN_32076853_380000/RConn3 -- 303_CN_44717036_380000_CN313937042/RConn3
  T_24493551_380000;110000_Ganderkesee/LConn1 -- 303_CN_44717036_380000_CN_24493551_380000/RConn1
  T_24493551_380000;110000_Ganderkesee/LConn2 -- 303_CN_44717036_380000_CN_24493551_380000/RConn2
  T_24493551_380000;110000_Ganderkesee/LConn3 -- 303_CN_44717036_380000_CN_24493551_380000/RConn3
  _CN_137602559_220000_CN29122363/RConn1 -- T_137602559_380000;220000;110000_Irsching/RConn1 -- L_137602559/LConn1
  _CN_137602559_220000_CN29122363/RConn2 -- T_137602559_380000;220000;110000_Irsching/RConn2 -- L_137602559/LConn2
  _CN_137602559_220000_CN29122363/RConn3 -- T_137602559_380000;220000;110000_Irsching/RConn3 -- L_137602559/LConn3
  T_137602559_380000;220000;110000_Irsching/LConn1 -- Irsching___Raitersaich_CN_137602559_380000_CN_24768051_380000/RConn1
  T_137602559_380000;220000;110000_Irsching/LConn2 -- Irsching___Raitersaich_CN_137602559_380000_CN_24768051_380000/RConn2
  T_137602559_380000;220000;110000_Irsching/LConn3 -- Irsching___Raitersaich_CN_137602559_380000_CN_24768051_380000/RConn3
  T_40621568_220000;110000_Brandenburg_West/LConn1 -- 324_CN_40621568_220000_CN_27149550_220000/RConn1
  T_40621568_220000;110000_Brandenburg_West/LConn2 -- 324_CN_40621568_220000_CN_27149550_220000/RConn2
  T_40621568_220000;110000_Brandenburg_West/LConn3 -- 324_CN_40621568_220000_CN_27149550_220000/RConn3
  220kV_Cappenberg_Nord+Elmenhorst_Süd_CN_138877959_220000_CN_42507488_220000/RConn1 -- T_138877959_220000_Rheinzink/LConn1 -- 220kV_Cappenberg_Nord+Elmenhorst_Süd_CN_138877959_220000_CN_24415232_220000/LConn1 -- 220kV_Cappenberg_Nord+Elmenhorst_Süd_CN_138877959_220000_CN_28452784_220000/RConn1
  220kV_Cappenberg_Nord+Elmenhorst_Süd_CN_138877959_220000_CN_42507488_220000/RConn2 -- T_138877959_220000_Rheinzink/LConn2 -- 220kV_Cappenberg_Nord+Elmenhorst_Süd_CN_138877959_220000_CN_24415232_220000/LConn2 -- 220kV_Cappenberg_Nord+Elmenhorst_Süd_CN_138877959_220000_CN_28452784_220000/RConn2
  220kV_Cappenberg_Nord+Elmenhorst_Süd_CN_138877959_220000_CN_42507488_220000/RConn3 -- T_138877959_220000_Rheinzink/LConn3 -- 220kV_Cappenberg_Nord+Elmenhorst_Süd_CN_138877959_220000_CN_24415232_220000/LConn3 -- 220kV_Cappenberg_Nord+Elmenhorst_Süd_CN_138877959_220000_CN_28452784_220000/RConn3
  T_24415232_220000;110000_Station_Elmenhorst/LConn1 -- 220kV_Cappenberg_Nord+Elmenhorst_Süd_CN_138877959_220000_CN_24415232_220000/RConn1
  T_24415232_220000;110000_Station_Elmenhorst/LConn2 -- 220kV_Cappenberg_Nord+Elmenhorst_Süd_CN_138877959_220000_CN_24415232_220000/RConn2
  T_24415232_220000;110000_Station_Elmenhorst/LConn3 -- 220kV_Cappenberg_Nord+Elmenhorst_Süd_CN_138877959_220000_CN_24415232_220000/RConn3
  LU_SIT_CN_24759324_220000_CN_133349218_220000/RConn1 -- T_24759324_220000;110000_Umspannwerk_Sittling/LConn1 -- Altheim___Sittling_CN_24759324_220000_CN_77694901_220000/RConn1 -- IN_SIT_CN_24759324_220000_CN_24768051_220000/LConn1
  LU_SIT_CN_24759324_220000_CN_133349218_220000/RConn2 -- T_24759324_220000;110000_Umspannwerk_Sittling/LConn2 -- Altheim___Sittling_CN_24759324_220000_CN_77694901_220000/RConn2 -- IN_SIT_CN_24759324_220000_CN_24768051_220000/LConn2
  LU_SIT_CN_24759324_220000_CN_133349218_220000/RConn3 -- T_24759324_220000;110000_Umspannwerk_Sittling/LConn3 -- Altheim___Sittling_CN_24759324_220000_CN_77694901_220000/RConn3 -- IN_SIT_CN_24759324_220000_CN_24768051_220000/LConn3
  IN_SIT_CN_24759324_220000_CN_24768051_220000/RConn1 -- T_24768051_380000;220000;110000_Ingolstadt/RConn1 -- L_24768051/LConn1
  IN_SIT_CN_24759324_220000_CN_24768051_220000/RConn2 -- T_24768051_380000;220000;110000_Ingolstadt/RConn2 -- L_24768051/LConn2
  IN_SIT_CN_24759324_220000_CN_24768051_220000/RConn3 -- T_24768051_380000;220000;110000_Ingolstadt/RConn3 -- L_24768051/LConn3
  T_22690852_220000;110000_Bocklemünd/LConn1 -- 220_kV_Bocklemünd_Nord|Süd_(Brauweiler)_CN_22690852_220000_CN_23084554_220000/RConn1
  T_22690852_220000;110000_Bocklemünd/LConn2 -- 220_kV_Bocklemünd_Nord|Süd_(Brauweiler)_CN_22690852_220000_CN_23084554_220000/RConn2
  T_22690852_220000;110000_Bocklemünd/LConn3 -- 220_kV_Bocklemünd_Nord|Süd_(Brauweiler)_CN_22690852_220000_CN_23084554_220000/RConn3
  T_109582315_380000;220000_Kernkraftwerk_Unterweser/LConn1 -- _CN_32076853_380000_CN_109582315_380000/RConn1
  T_109582315_380000;220000_Kernkraftwerk_Unterweser/LConn2 -- _CN_32076853_380000_CN_109582315_380000/RConn2
  T_109582315_380000;220000_Kernkraftwerk_Unterweser/LConn3 -- _CN_32076853_380000_CN_109582315_380000/RConn3
  302_CN_32076853_220000_CN_173178563_220000/RConn1 -- T_32076853_380000;220000;110000_Unterweser/RConn1 -- L_32076853/LConn1
  302_CN_32076853_220000_CN_173178563_220000/RConn2 -- T_32076853_380000;220000;110000_Unterweser/RConn2 -- L_32076853/LConn2
  302_CN_32076853_220000_CN_173178563_220000/RConn3 -- T_32076853_380000;220000;110000_Unterweser/RConn3 -- L_32076853/LConn3
  T_153328698_380000_Gemeinschaftskraftwerk_Neckarwestheim_2/LConn1 -- _CN_153328698_380000_CN23547196/RConn1
  T_153328698_380000_Gemeinschaftskraftwerk_Neckarwestheim_2/LConn2 -- _CN_153328698_380000_CN23547196/RConn2
  T_153328698_380000_Gemeinschaftskraftwerk_Neckarwestheim_2/LConn3 -- _CN_153328698_380000_CN23547196/RConn3
  T_154110135_380000_Philippsburg_380_kV/LConn1 -- Daxlanden___Philippsburg_CN_154110135_380000_CN161909939/RConn1
  T_154110135_380000_Philippsburg_380_kV/LConn2 -- Daxlanden___Philippsburg_CN_154110135_380000_CN161909939/RConn2
  T_154110135_380000_Philippsburg_380_kV/LConn3 -- Daxlanden___Philippsburg_CN_154110135_380000_CN161909939/RConn3
  903;_904_CN_11500045_380000_CN_46615737_380000/LConn1 -- T_11500045_380000_380_kV_Kabel_Terminal_Berlin/LConn1 -- 903;_904_CN_11500045_380000_CN_43163132_380000/RConn1
  903;_904_CN_11500045_380000_CN_46615737_380000/LConn2 -- T_11500045_380000_380_kV_Kabel_Terminal_Berlin/LConn2 -- 903;_904_CN_11500045_380000_CN_43163132_380000/RConn2
  903;_904_CN_11500045_380000_CN_46615737_380000/LConn3 -- T_11500045_380000_380_kV_Kabel_Terminal_Berlin/LConn3 -- 903;_904_CN_11500045_380000_CN_43163132_380000/RConn3
  903;_904_CN_11500045_380000_CN_46615737_380000/RConn1 -- T_46615737_380000;110000_Umspannwerk_Charlottenburg/LConn1 -- 380_kV_Transversale_Berlin_CN_46615737_380000_CN_30303506_380000/LConn1
  903;_904_CN_11500045_380000_CN_46615737_380000/RConn2 -- T_46615737_380000;110000_Umspannwerk_Charlottenburg/LConn2 -- 380_kV_Transversale_Berlin_CN_46615737_380000_CN_30303506_380000/LConn2
  903;_904_CN_11500045_380000_CN_46615737_380000/RConn3 -- T_46615737_380000;110000_Umspannwerk_Charlottenburg/LConn3 -- 380_kV_Transversale_Berlin_CN_46615737_380000_CN_30303506_380000/LConn3
  T_150267232_220000_LMG/LConn1 -- 220kV_LMG_West_CN_24921206_220000_CN_150267232_220000/RConn1
  T_150267232_220000_LMG/LConn2 -- 220kV_LMG_West_CN_24921206_220000_CN_150267232_220000/RConn2
  T_150267232_220000_LMG/LConn3 -- 220kV_LMG_West_CN_24921206_220000_CN_150267232_220000/RConn3
  T_42423415_220000;110000_Station_Meckenheim/LConn1 -- 220_kV_Berggeist_West;_Nette_Ost_CN_42423415_220000_CN_395847307_220000/RConn1
  T_42423415_220000;110000_Station_Meckenheim/LConn2 -- 220_kV_Berggeist_West;_Nette_Ost_CN_42423415_220000_CN_395847307_220000/RConn2
  T_42423415_220000;110000_Station_Meckenheim/LConn3 -- 220_kV_Berggeist_West;_Nette_Ost_CN_42423415_220000_CN_395847307_220000/RConn3
  _CN_42681484_380000_CN_274630377_380000/LConn1 -- T_42681484_380000;110000_Vörden/LConn1 -- _CN_42681484_380000_CN_24413992_380000/RConn1
  _CN_42681484_380000_CN_274630377_380000/LConn2 -- T_42681484_380000;110000_Vörden/LConn2 -- _CN_42681484_380000_CN_24413992_380000/RConn2
  _CN_42681484_380000_CN_274630377_380000/LConn3 -- T_42681484_380000;110000_Vörden/LConn3 -- _CN_42681484_380000_CN_24413992_380000/RConn3
  _CN_42681484_380000_CN_274630377_380000/RConn1 -- T_274630377_380000;220000;110000_Umspannanlage_Würgassen/LConn1 -- _CN_274630377_380000_CN_156960655_380000/LConn1
  _CN_42681484_380000_CN_274630377_380000/RConn2 -- T_274630377_380000;220000;110000_Umspannanlage_Würgassen/LConn2 -- _CN_274630377_380000_CN_156960655_380000/LConn2
  _CN_42681484_380000_CN_274630377_380000/RConn3 -- T_274630377_380000;220000;110000_Umspannanlage_Würgassen/LConn3 -- _CN_274630377_380000_CN_156960655_380000/LConn3
  _CN_128277645_220000_CN_152219167_220000/LConn1 -- T_128277645_380000;220000;110000_Umspannwerk_Remptendorf/RConn1 -- _CN_128277645_220000_CN136858836/LConn1 -- L_128277645/LConn1
  _CN_128277645_220000_CN_152219167_220000/LConn2 -- T_128277645_380000;220000;110000_Umspannwerk_Remptendorf/RConn2 -- _CN_128277645_220000_CN136858836/LConn2 -- L_128277645/LConn2
  _CN_128277645_220000_CN_152219167_220000/LConn3 -- T_128277645_380000;220000;110000_Umspannwerk_Remptendorf/RConn3 -- _CN_128277645_220000_CN136858836/LConn3 -- L_128277645/LConn3
  T_152219167_220000_Stahlwerk_Thüringen/LConn1 -- _CN_128277645_220000_CN_152219167_220000/RConn1
  T_152219167_220000_Stahlwerk_Thüringen/LConn2 -- _CN_128277645_220000_CN_152219167_220000/RConn2
  T_152219167_220000_Stahlwerk_Thüringen/LConn3 -- _CN_128277645_220000_CN_152219167_220000/RConn3
  G_136858836_Pumpspeicherkraftwerk_Hohenwarte_II/RConn1 -- _CN_128277645_220000_CN136858836/RConn1
  G_136858836_Pumpspeicherkraftwerk_Hohenwarte_II/RConn2 -- _CN_128277645_220000_CN136858836/RConn2
  G_136858836_Pumpspeicherkraftwerk_Hohenwarte_II/RConn3 -- _CN_128277645_220000_CN136858836/RConn3
  T_156673637_380000;220000;110000_Umspannwerk_Weida/LConn1 -- 574_Remptendorf___Röhrsdorf;_573_Remptendorf___Weida_CN_128277645_380000_CN_156673637_380000/RConn1
  T_156673637_380000;220000;110000_Umspannwerk_Weida/LConn2 -- 574_Remptendorf___Röhrsdorf;_573_Remptendorf___Weida_CN_128277645_380000_CN_156673637_380000/RConn2
  T_156673637_380000;220000;110000_Umspannwerk_Weida/LConn3 -- 574_Remptendorf___Röhrsdorf;_573_Remptendorf___Weida_CN_128277645_380000_CN_156673637_380000/RConn3
  _CN_24536211_380000_CN_202747445_380000/RConn1 -- T_24536211_380000;110000_Umspannwerk_Aßlar/LConn1 -- _CN_24536211_380000_CN_152403632_380000/RConn1 -- _CN_24536211_380000_CN_24536328_380000/LConn1
  _CN_24536211_380000_CN_202747445_380000/RConn2 -- T_24536211_380000;110000_Umspannwerk_Aßlar/LConn2 -- _CN_24536211_380000_CN_152403632_380000/RConn2 -- _CN_24536211_380000_CN_24536328_380000/LConn2
  _CN_24536211_380000_CN_202747445_380000/RConn3 -- T_24536211_380000;110000_Umspannwerk_Aßlar/LConn3 -- _CN_24536211_380000_CN_152403632_380000/RConn3 -- _CN_24536211_380000_CN_24536328_380000/LConn3
  T_24536328_380000;110000_Dillenburg/LConn1 -- _CN_24536211_380000_CN_24536328_380000/RConn1
  T_24536328_380000;110000_Dillenburg/LConn2 -- _CN_24536211_380000_CN_24536328_380000/RConn2
  T_24536328_380000;110000_Dillenburg/LConn3 -- _CN_24536211_380000_CN_24536328_380000/RConn3
  T_23161029_220000;110000_Umspannwerk_Taucha/LConn1 -- _CN_23161029_220000_CN_32843531_220000/LConn1
  T_23161029_220000;110000_Umspannwerk_Taucha/LConn2 -- _CN_23161029_220000_CN_32843531_220000/LConn2
  T_23161029_220000;110000_Umspannwerk_Taucha/LConn3 -- _CN_23161029_220000_CN_32843531_220000/LConn3
  _CN_23161029_220000_CN_32843531_220000/RConn1 -- T_32843531_380000;220000;110000_Eula/RConn1 -- _CN_22879599_220000_CN_32843531_220000/RConn1 -- L_32843531/LConn1 -- 203_Eula_CN_23117075_220000_CN_32843531_220000/RConn1
  _CN_23161029_220000_CN_32843531_220000/RConn2 -- T_32843531_380000;220000;110000_Eula/RConn2 -- _CN_22879599_220000_CN_32843531_220000/RConn2 -- L_32843531/LConn2 -- 203_Eula_CN_23117075_220000_CN_32843531_220000/RConn2
  _CN_23161029_220000_CN_32843531_220000/RConn3 -- T_32843531_380000;220000;110000_Eula/RConn3 -- _CN_22879599_220000_CN_32843531_220000/RConn3 -- L_32843531/LConn3 -- 203_Eula_CN_23117075_220000_CN_32843531_220000/RConn3
  T_201153704_380000;220000_Kraftwerkschaltanlage_Knapsack_1/LConn1 -- 380_kV_Knapsack_1a_CN_201153704_380000_CN_22765517_380000/RConn1
  T_201153704_380000;220000_Kraftwerkschaltanlage_Knapsack_1/LConn2 -- 380_kV_Knapsack_1a_CN_201153704_380000_CN_22765517_380000/RConn2
  T_201153704_380000;220000_Kraftwerkschaltanlage_Knapsack_1/LConn3 -- 380_kV_Knapsack_1a_CN_201153704_380000_CN_22765517_380000/RConn3
  T_24478889_220000;110000_Station_Walsum/LConn1 -- 220kV_Beeck_Tr211+212_CN_24478889_220000_CN26623135/RConn1
  T_24478889_220000;110000_Station_Walsum/LConn2 -- 220kV_Beeck_Tr211+212_CN_24478889_220000_CN26623135/RConn2
  T_24478889_220000;110000_Station_Walsum/LConn3 -- 220kV_Beeck_Tr211+212_CN_24478889_220000_CN26623135/RConn3
  380_kV_Transversale_Berlin_CN_46615737_380000_CN_30303506_380000/RConn1 -- T_30303506_380000;110000_Berlin_Mitte/LConn1 -- 380_kV_Transversale_Berlin_CN_30954714_380000_CN_30303506_380000/RConn1
  380_kV_Transversale_Berlin_CN_46615737_380000_CN_30303506_380000/RConn2 -- T_30303506_380000;110000_Berlin_Mitte/LConn2 -- 380_kV_Transversale_Berlin_CN_30954714_380000_CN_30303506_380000/RConn2
  380_kV_Transversale_Berlin_CN_46615737_380000_CN_30303506_380000/RConn3 -- T_30303506_380000;110000_Berlin_Mitte/LConn3 -- 380_kV_Transversale_Berlin_CN_30954714_380000_CN_30303506_380000/RConn3
  380_kV_Gilzem_Ost;_Uchtelfangen_Ost_CN_42097854_380000_CN_54359256_380000/RConn1 -- T_42097854_380000;110000_Station_Osburg/LConn1 -- 380_kV_Gilzem_Ost;_Uchtelfangen_Ost_CN_42097854_380000_CN_151967290_380000/LConn1
  380_kV_Gilzem_Ost;_Uchtelfangen_Ost_CN_42097854_380000_CN_54359256_380000/RConn2 -- T_42097854_380000;110000_Station_Osburg/LConn2 -- 380_kV_Gilzem_Ost;_Uchtelfangen_Ost_CN_42097854_380000_CN_151967290_380000/LConn2
  380_kV_Gilzem_Ost;_Uchtelfangen_Ost_CN_42097854_380000_CN_54359256_380000/RConn3 -- T_42097854_380000;110000_Station_Osburg/LConn3 -- 380_kV_Gilzem_Ost;_Uchtelfangen_Ost_CN_42097854_380000_CN_151967290_380000/LConn3
  380_kV_Gilzem_Ost;_Uchtelfangen_Ost_CN_42097854_380000_CN_151967290_380000/RConn1 -- T_151967290_380000;220000;110000_Station_Niederstedem/LConn1 -- _CN_151967290_380000_CN_32675761_380000/LConn1 -- _CN_151967290_380000_CN_26593929_380000/RConn1
  380_kV_Gilzem_Ost;_Uchtelfangen_Ost_CN_42097854_380000_CN_151967290_380000/RConn2 -- T_151967290_380000;220000;110000_Station_Niederstedem/LConn2 -- _CN_151967290_380000_CN_32675761_380000/LConn2 -- _CN_151967290_380000_CN_26593929_380000/RConn2
  380_kV_Gilzem_Ost;_Uchtelfangen_Ost_CN_42097854_380000_CN_151967290_380000/RConn3 -- T_151967290_380000;220000;110000_Station_Niederstedem/LConn3 -- _CN_151967290_380000_CN_32675761_380000/LConn3 -- _CN_151967290_380000_CN_26593929_380000/RConn3
  T_83916207_220000;110000_Elverlingsen/LConn1 -- 220kV_Nordleitung_CN_24667346_220000_CN_83916207_220000/RConn1
  T_83916207_220000;110000_Elverlingsen/LConn2 -- 220kV_Nordleitung_CN_24667346_220000_CN_83916207_220000/RConn2
  T_83916207_220000;110000_Elverlingsen/LConn3 -- 220kV_Nordleitung_CN_24667346_220000_CN_83916207_220000/RConn3
  _CN_54359256_380000_CN115145869/RConn1 -- G_115145869_Kraftwerk_Ensdorf/RConn1 -- 220_kV_CN_82773910_220000_CN115145869/LConn1 -- _CN_82773910_380000_CN115145869/LConn1
  _CN_54359256_380000_CN115145869/RConn2 -- G_115145869_Kraftwerk_Ensdorf/RConn2 -- 220_kV_CN_82773910_220000_CN115145869/LConn2 -- _CN_82773910_380000_CN115145869/LConn2
  _CN_54359256_380000_CN115145869/RConn3 -- G_115145869_Kraftwerk_Ensdorf/RConn3 -- 220_kV_CN_82773910_220000_CN115145869/LConn3 -- _CN_82773910_380000_CN115145869/LConn3
  _CN_54359256_220000_CN_100812630_220000/RConn1 -- T_100812630_220000;110000_/LConn1 -- _CN_100812630_220000_CN30425117/LConn1
  _CN_54359256_220000_CN_100812630_220000/RConn2 -- T_100812630_220000;110000_/LConn2 -- _CN_100812630_220000_CN30425117/LConn2
  _CN_54359256_220000_CN_100812630_220000/RConn3 -- T_100812630_220000;110000_/LConn3 -- _CN_100812630_220000_CN30425117/LConn3
  _CN_54359256_220000_CN30425117/RConn1 -- G_30425117_Kraftwerk_Weiher/RConn1 -- _CN_100812630_220000_CN30425117/RConn1
  _CN_54359256_220000_CN30425117/RConn2 -- G_30425117_Kraftwerk_Weiher/RConn2 -- _CN_100812630_220000_CN30425117/RConn2
  _CN_54359256_220000_CN30425117/RConn3 -- G_30425117_Kraftwerk_Weiher/RConn3 -- _CN_100812630_220000_CN30425117/RConn3
  T_30309989_220000_Hennigsdorf/LConn1 -- 294_CN_27149550_220000_CN_30309989_220000/RConn1
  T_30309989_220000_Hennigsdorf/LConn2 -- 294_CN_27149550_220000_CN_30309989_220000/RConn2
  T_30309989_220000_Hennigsdorf/LConn3 -- 294_CN_27149550_220000_CN_30309989_220000/RConn3
  G_101400025_Kraftwerk_Moorburg/RConn1 -- _CN_11285720_380000_CN101400025/RConn1
  G_101400025_Kraftwerk_Moorburg/RConn2 -- _CN_11285720_380000_CN101400025/RConn2
  G_101400025_Kraftwerk_Moorburg/RConn3 -- _CN_11285720_380000_CN101400025/RConn3
  T_35763481_380000;110000_Station_Witten/LConn1 -- Trafo_411_CN_35763480_380000_CN_35763481_380000/RConn1
  T_35763481_380000;110000_Station_Witten/LConn2 -- Trafo_411_CN_35763480_380000_CN_35763481_380000/RConn2
  T_35763481_380000;110000_Station_Witten/LConn3 -- Trafo_411_CN_35763480_380000_CN_35763481_380000/RConn3
  T_24479003_220000_Station_Möllen/LConn1 -- _CN_24479003_380000_CN401873466/RConn1
  T_24479003_220000_Station_Möllen/LConn2 -- _CN_24479003_380000_CN401873466/RConn2
  T_24479003_220000_Station_Möllen/LConn3 -- _CN_24479003_380000_CN401873466/RConn3
  _CN_24479003_220000_CN401873466/RConn1 -- T_24479003_220000_Station_Möllen/RConn1 -- L_24479003/LConn1
  _CN_24479003_220000_CN401873466/RConn2 -- T_24479003_220000_Station_Möllen/RConn2 -- L_24479003/LConn2
  _CN_24479003_220000_CN401873466/RConn3 -- T_24479003_220000_Station_Möllen/RConn3 -- L_24479003/LConn3
  220kV_Gersteinwerk_I2_CN_42507488_220000_CN33883956/RConn1 -- G_33883956_/RConn1 -- 380kV_Gersteinwerk_K2_CN_42507488_380000_CN33883956/RConn1
  220kV_Gersteinwerk_I2_CN_42507488_220000_CN33883956/RConn2 -- G_33883956_/RConn2 -- 380kV_Gersteinwerk_K2_CN_42507488_380000_CN33883956/RConn2
  220kV_Gersteinwerk_I2_CN_42507488_220000_CN33883956/RConn3 -- G_33883956_/RConn3 -- 380kV_Gersteinwerk_K2_CN_42507488_380000_CN33883956/RConn3
  202_UW_HH_Nord_UW_Itzehoe_West_CN_60032354_220000_CN_28008024_220000/RConn1 -- T_60032354_220000;110000_Itzehoe_West/LConn1 -- 202_UW_HH_Nord_UW_Itzehoe_West_CN_60032354_220000_CN275650140/RConn1 -- _CN_60032354_220000_CN55015415/RConn1
  202_UW_HH_Nord_UW_Itzehoe_West_CN_60032354_220000_CN_28008024_220000/RConn2 -- T_60032354_220000;110000_Itzehoe_West/LConn2 -- 202_UW_HH_Nord_UW_Itzehoe_West_CN_60032354_220000_CN275650140/RConn2 -- _CN_60032354_220000_CN55015415/RConn2
  202_UW_HH_Nord_UW_Itzehoe_West_CN_60032354_220000_CN_28008024_220000/RConn3 -- T_60032354_220000;110000_Itzehoe_West/LConn3 -- 202_UW_HH_Nord_UW_Itzehoe_West_CN_60032354_220000_CN275650140/RConn3 -- _CN_60032354_220000_CN55015415/RConn3
  T_48428875_380000;110000_EnBW_Umspannwerk_Endersbach/LConn1 -- AL1_EDS_380_kV_CN_48428875_380000_CN25973419/RConn1
  T_48428875_380000;110000_EnBW_Umspannwerk_Endersbach/LConn2 -- AL1_EDS_380_kV_CN_48428875_380000_CN25973419/RConn2
  T_48428875_380000;110000_EnBW_Umspannwerk_Endersbach/LConn3 -- AL1_EDS_380_kV_CN_48428875_380000_CN25973419/RConn3
  220_kV_Neurath_1a_CN_27919734_220000_CN_95434457_220000/RConn1 -- T_95434457_380000;220000;110000_KW_Neurath/RConn1 -- L_95434457/LConn1
  220_kV_Neurath_1a_CN_27919734_220000_CN_95434457_220000/RConn2 -- T_95434457_380000;220000;110000_KW_Neurath/RConn2 -- L_95434457/LConn2
  220_kV_Neurath_1a_CN_27919734_220000_CN_95434457_220000/RConn3 -- T_95434457_380000;220000;110000_KW_Neurath/RConn3 -- L_95434457/LConn3
  T_156676050_220000;110000_Umspannanlage_Heidelberg_Süd/LConn1 -- _CN_207248812_220000_CN_156676050_220000/RConn1
  T_156676050_220000;110000_Umspannanlage_Heidelberg_Süd/LConn2 -- _CN_207248812_220000_CN_156676050_220000/RConn2
  T_156676050_220000;110000_Umspannanlage_Heidelberg_Süd/LConn3 -- _CN_207248812_220000_CN_156676050_220000/RConn3
  _CN_87952821_220000_CN_33148774_220000/RConn1 -- T_87952821_380000;220000;110000;20000_Flensburg/RConn1 -- L_87952821/LConn1
  _CN_87952821_220000_CN_33148774_220000/RConn2 -- T_87952821_380000;220000;110000;20000_Flensburg/RConn2 -- L_87952821/LConn2
  _CN_87952821_220000_CN_33148774_220000/RConn3 -- T_87952821_380000;220000;110000;20000_Flensburg/RConn3 -- L_87952821/LConn3
  T_31762305_220000;110000_Station_Norf/LConn1 -- 220_kV_Frimmersdorf_5e;_Zons_Nord_CN_49577401_220000_CN_31762305_220000/RConn1
  T_31762305_220000;110000_Station_Norf/LConn2 -- 220_kV_Frimmersdorf_5e;_Zons_Nord_CN_49577401_220000_CN_31762305_220000/RConn2
  T_31762305_220000;110000_Station_Norf/LConn3 -- 220_kV_Frimmersdorf_5e;_Zons_Nord_CN_49577401_220000_CN_31762305_220000/RConn3
  380kV_Voerde_B_CN_76185022_380000_CN401873466/RConn1 -- T_76185022_380000_Station_Zensenbusch/LConn1 -- _CN_76185022_380000_CN26623135/RConn1
  380kV_Voerde_B_CN_76185022_380000_CN401873466/RConn2 -- T_76185022_380000_Station_Zensenbusch/LConn2 -- _CN_76185022_380000_CN26623135/RConn2
  380kV_Voerde_B_CN_76185022_380000_CN401873466/RConn3 -- T_76185022_380000_Station_Zensenbusch/LConn3 -- _CN_76185022_380000_CN26623135/RConn3
  T_37721677_380000;110000_EnBW_Umspannwerk_Altbach_1/LConn1 -- AL1_BZW_380_kV_CN_37721677_380000_CN25973419/RConn1
  T_37721677_380000;110000_EnBW_Umspannwerk_Altbach_1/LConn2 -- AL1_BZW_380_kV_CN_37721677_380000_CN25973419/RConn2
  T_37721677_380000;110000_EnBW_Umspannwerk_Altbach_1/LConn3 -- AL1_BZW_380_kV_CN_37721677_380000_CN25973419/RConn3
  G_218161891_Kraftwerk_Schkopau/RConn1 -- _CN_29713902_380000_CN218161891/RConn1
  G_218161891_Kraftwerk_Schkopau/RConn2 -- _CN_29713902_380000_CN218161891/RConn2
  G_218161891_Kraftwerk_Schkopau/RConn3 -- _CN_29713902_380000_CN218161891/RConn3
  G_185569568_Heizkraftwerk_Reuter_West/RConn1 -- _CN_43163132_380000_CN185569568/RConn1
  G_185569568_Heizkraftwerk_Reuter_West/RConn2 -- _CN_43163132_380000_CN185569568/RConn2
  G_185569568_Heizkraftwerk_Reuter_West/RConn3 -- _CN_43163132_380000_CN185569568/RConn3
  T_154869247_220000_/LConn1 -- _CN_154869247_220000_CN_395847307_220000/RConn1
  T_154869247_220000_/LConn2 -- _CN_154869247_220000_CN_395847307_220000/RConn2
  T_154869247_220000_/LConn3 -- _CN_154869247_220000_CN_395847307_220000/RConn3
  Leitung_2008_CN_28921360_220000_CN-2022229/RConn1 -- T_28921360_220000_Umspannwerk_Kraftwerk_Robert_Frank/LConn1 -- Leitung_3004_CN_28921360_220000_CN_27739871_220000/LConn1
  Leitung_2008_CN_28921360_220000_CN-2022229/RConn2 -- T_28921360_220000_Umspannwerk_Kraftwerk_Robert_Frank/LConn2 -- Leitung_3004_CN_28921360_220000_CN_27739871_220000/LConn2
  Leitung_2008_CN_28921360_220000_CN-2022229/RConn3 -- T_28921360_220000_Umspannwerk_Kraftwerk_Robert_Frank/LConn3 -- Leitung_3004_CN_28921360_220000_CN_27739871_220000/LConn3
  Leitung_3004_CN_28921360_220000_CN_27739871_220000/RConn1 -- T_27739871_380000;220000_Landesbergen/RConn1 -- L_27739871/LConn1
  Leitung_3004_CN_28921360_220000_CN_27739871_220000/RConn2 -- T_27739871_380000;220000_Landesbergen/RConn2 -- L_27739871/LConn2
  Leitung_3004_CN_28921360_220000_CN_27739871_220000/RConn3 -- T_27739871_380000;220000_Landesbergen/RConn3 -- L_27739871/LConn3
  Dellmensingen___Obermooweiler;Dellmensingen_Ost_CN_41389594_380000_CN_31131320_380000/RConn1 -- T_31131320_380000_Umspannwerk_Obermooweiler/LConn1 -- _CN_31131320_380000_CN_31131325_380000/LConn1
  Dellmensingen___Obermooweiler;Dellmensingen_Ost_CN_41389594_380000_CN_31131320_380000/RConn2 -- T_31131320_380000_Umspannwerk_Obermooweiler/LConn2 -- _CN_31131320_380000_CN_31131325_380000/LConn2
  Dellmensingen___Obermooweiler;Dellmensingen_Ost_CN_41389594_380000_CN_31131320_380000/RConn3 -- T_31131320_380000_Umspannwerk_Obermooweiler/LConn3 -- _CN_31131320_380000_CN_31131325_380000/LConn3
  T_97857512_220000_/LConn1 -- _CN_28227099_220000_CN_97857512_220000/RConn1
  T_97857512_220000_/LConn2 -- _CN_28227099_220000_CN_97857512_220000/RConn2
  T_97857512_220000_/LConn3 -- _CN_28227099_220000_CN_97857512_220000/RConn3
  T_42872354_220000_Huntorf/LConn1 -- Huntorf_CN_42872354_220000_CN42872353/LConn1
  T_42872354_220000_Huntorf/LConn2 -- Huntorf_CN_42872354_220000_CN42872353/LConn2
  T_42872354_220000_Huntorf/LConn3 -- Huntorf_CN_42872354_220000_CN42872353/LConn3
  G_42872353_Druckluftspeicher__und_Gasturbinenkraftwerk_Huntorf/RConn1 -- Huntorf_CN_42872354_220000_CN42872353/RConn1
  G_42872353_Druckluftspeicher__und_Gasturbinenkraftwerk_Huntorf/RConn2 -- Huntorf_CN_42872354_220000_CN42872353/RConn2
  G_42872353_Druckluftspeicher__und_Gasturbinenkraftwerk_Huntorf/RConn3 -- Huntorf_CN_42872354_220000_CN42872353/RConn3
  _CN_23881272_220000_CN_42411962_220000/RConn1 -- T_23881272_220000;110000_Dörnigheim_220_kV/LConn1 -- _CN_23881272_220000_CN_4826893_220000/LConn1
  _CN_23881272_220000_CN_42411962_220000/RConn2 -- T_23881272_220000;110000_Dörnigheim_220_kV/LConn2 -- _CN_23881272_220000_CN_4826893_220000/LConn2
  _CN_23881272_220000_CN_42411962_220000/RConn3 -- T_23881272_220000;110000_Dörnigheim_220_kV/LConn3 -- _CN_23881272_220000_CN_4826893_220000/LConn3
  T_4826893_220000;110000_Umspannwerk_Frankfurt_Nord/LConn1 -- _CN_23881272_220000_CN_4826893_220000/RConn1
  T_4826893_220000;110000_Umspannwerk_Frankfurt_Nord/LConn2 -- _CN_23881272_220000_CN_4826893_220000/RConn2
  T_4826893_220000;110000_Umspannwerk_Frankfurt_Nord/LConn3 -- _CN_23881272_220000_CN_4826893_220000/RConn3
  T_32675761_380000;110000_Station_Dahlem/LConn1 -- _CN_151967290_380000_CN_32675761_380000/RConn1
  T_32675761_380000;110000_Station_Dahlem/LConn2 -- _CN_151967290_380000_CN_32675761_380000/RConn2
  T_32675761_380000;110000_Station_Dahlem/LConn3 -- _CN_151967290_380000_CN_32675761_380000/RConn3
  G_125808869_Kraftwerk_Hamborn_Block_5/RConn1 -- _CN_35833442_220000_CN125808869/RConn1
  G_125808869_Kraftwerk_Hamborn_Block_5/RConn2 -- _CN_35833442_220000_CN125808869/RConn2
  G_125808869_Kraftwerk_Hamborn_Block_5/RConn3 -- _CN_35833442_220000_CN125808869/RConn3
  _CN_156673636_380000_CN_156960655_380000/RConn1 -- T_156960655_380000;110000_Umspannwerk_Bergshausen/LConn1 -- _CN_274630377_380000_CN_156960655_380000/RConn1
  _CN_156673636_380000_CN_156960655_380000/RConn2 -- T_156960655_380000;110000_Umspannwerk_Bergshausen/LConn2 -- _CN_274630377_380000_CN_156960655_380000/RConn2
  _CN_156673636_380000_CN_156960655_380000/RConn3 -- T_156960655_380000;110000_Umspannwerk_Bergshausen/LConn3 -- _CN_274630377_380000_CN_156960655_380000/RConn3
  T_41072584_380000_UW_Waldeck/LConn1 -- Leitung_3212;Leitung_3213_CN_156673636_380000_CN_41072584_380000/RConn1
  T_41072584_380000_UW_Waldeck/LConn2 -- Leitung_3212;Leitung_3213_CN_156673636_380000_CN_41072584_380000/RConn2
  T_41072584_380000_UW_Waldeck/LConn3 -- Leitung_3212;Leitung_3213_CN_156673636_380000_CN_41072584_380000/RConn3
  Herbertingen___Grünkraut_CN_25306752_380000_CN_31131325_380000/RConn1 -- T_31131325_380000;110000_380kV_Umspannwerk_Grünkraut/LConn1 -- _CN_31131320_380000_CN_31131325_380000/RConn1
  Herbertingen___Grünkraut_CN_25306752_380000_CN_31131325_380000/RConn2 -- T_31131325_380000;110000_380kV_Umspannwerk_Grünkraut/LConn2 -- _CN_31131320_380000_CN_31131325_380000/RConn2
  Herbertingen___Grünkraut_CN_25306752_380000_CN_31131325_380000/RConn3 -- T_31131325_380000;110000_380kV_Umspannwerk_Grünkraut/LConn3 -- _CN_31131320_380000_CN_31131325_380000/RConn3
  T_106976898_220000_Saarstahl/LConn1 -- _CN_106976898_220000_CN_31135714_220000/LConn1
  T_106976898_220000_Saarstahl/LConn2 -- _CN_106976898_220000_CN_31135714_220000/LConn2
  T_106976898_220000_Saarstahl/LConn3 -- _CN_106976898_220000_CN_31135714_220000/LConn3
  T_31135714_220000;110000_Umspannwerk_Heinitz/LConn1 -- _CN_106976898_220000_CN_31135714_220000/RConn1
  T_31135714_220000;110000_Umspannwerk_Heinitz/LConn2 -- _CN_106976898_220000_CN_31135714_220000/RConn2
  T_31135714_220000;110000_Umspannwerk_Heinitz/LConn3 -- _CN_106976898_220000_CN_31135714_220000/RConn3
  T_25992879_380000;110000_Siersdorf/LConn1 -- _CN_25992879_380000_CN_26593929_380000/RConn1
  T_25992879_380000;110000_Siersdorf/LConn2 -- _CN_25992879_380000_CN_26593929_380000/RConn2
  T_25992879_380000;110000_Siersdorf/LConn3 -- _CN_25992879_380000_CN_26593929_380000/RConn3
  T_157449983_380000_/LConn1 -- Emsland_D1|D2|D0_CN_157449983_380000_CN49339874/RConn1
  T_157449983_380000_/LConn2 -- Emsland_D1|D2|D0_CN_157449983_380000_CN49339874/RConn2
  T_157449983_380000_/LConn3 -- Emsland_D1|D2|D0_CN_157449983_380000_CN49339874/RConn3
  T_157421330_220000_Atlantic/LConn1 -- Maade_gelb_CN_157421330_220000_CN_23744346_220000/RConn1
  T_157421330_220000_Atlantic/LConn2 -- Maade_gelb_CN_157421330_220000_CN_23744346_220000/RConn2
  T_157421330_220000_Atlantic/LConn3 -- Maade_gelb_CN_157421330_220000_CN_23744346_220000/RConn3
  G_26470129_Uniper_Kraftwerk_Wilhelmshaven/RConn1 -- 300_CN_23744346_220000_CN26470129/RConn1
  G_26470129_Uniper_Kraftwerk_Wilhelmshaven/RConn2 -- 300_CN_23744346_220000_CN26470129/RConn2
  G_26470129_Uniper_Kraftwerk_Wilhelmshaven/RConn3 -- 300_CN_23744346_220000_CN26470129/RConn3
  220_kV_CN_82773910_220000_CN115145869/RConn1 -- T_82773910_380000;220000;110000_Umspannanlage_Ensdorf/RConn1 -- L_82773910/LConn1
  220_kV_CN_82773910_220000_CN115145869/RConn2 -- T_82773910_380000;220000;110000_Umspannanlage_Ensdorf/RConn2 -- L_82773910/LConn2
  220_kV_CN_82773910_220000_CN115145869/RConn3 -- T_82773910_380000;220000;110000_Umspannanlage_Ensdorf/RConn3 -- L_82773910/LConn3
  T_82773910_380000;220000;110000_Umspannanlage_Ensdorf/LConn1 -- _CN_82773910_380000_CN115145869/RConn1
  T_82773910_380000;220000;110000_Umspannanlage_Ensdorf/LConn2 -- _CN_82773910_380000_CN115145869/RConn2
  T_82773910_380000;220000;110000_Umspannanlage_Ensdorf/LConn3 -- _CN_82773910_380000_CN115145869/RConn3
  G_-536706_Kraftwerk_Knepper/RConn1 -- 220kV_Knepper_C_CN_28452784_220000_CN-536706/RConn1
  G_-536706_Kraftwerk_Knepper/RConn2 -- 220kV_Knepper_C_CN_28452784_220000_CN-536706/RConn2
  G_-536706_Kraftwerk_Knepper/RConn3 -- 220kV_Knepper_C_CN_28452784_220000_CN-536706/RConn3
  G_11341038_Kraftwerk_Jänschwalde/RConn1 -- _CN_23025610_380000_CN11341038/RConn1
  G_11341038_Kraftwerk_Jänschwalde/RConn2 -- _CN_23025610_380000_CN11341038/RConn2
  G_11341038_Kraftwerk_Jänschwalde/RConn3 -- _CN_23025610_380000_CN11341038/RConn3
  T_23816140_220000;110000_Lahe/LConn1 -- _CN_23816140_220000_CN23681460/RConn1
  T_23816140_220000;110000_Lahe/LConn2 -- _CN_23816140_220000_CN23681460/RConn2
  T_23816140_220000;110000_Lahe/LConn3 -- _CN_23816140_220000_CN23681460/RConn3
  G_239364386_Statkraft_Kraftwerk_Knapsack_II/RConn1 -- _CN_22765517_380000_CN239364386/RConn1
  G_239364386_Statkraft_Kraftwerk_Knapsack_II/RConn2 -- _CN_22765517_380000_CN239364386/RConn2
  G_239364386_Statkraft_Kraftwerk_Knapsack_II/RConn3 -- _CN_22765517_380000_CN239364386/RConn3
  _CN_275138524_380000_CN275138522/LConn1 -- T_275138524_380000;110000_Schaltanlage_Datteln_4/LConn1 -- _CN_275138524_380000_CN109504648/RConn1 -- _CN_275138524_380000_CN275138520/LConn1 -- _CN_275138524_380000_CN275138521/LConn1 -- _CN_275138524_380000_CN275138523/LConn1
  _CN_275138524_380000_CN275138522/LConn2 -- T_275138524_380000;110000_Schaltanlage_Datteln_4/LConn2 -- _CN_275138524_380000_CN109504648/RConn2 -- _CN_275138524_380000_CN275138520/LConn2 -- _CN_275138524_380000_CN275138521/LConn2 -- _CN_275138524_380000_CN275138523/LConn2
  _CN_275138524_380000_CN275138522/LConn3 -- T_275138524_380000;110000_Schaltanlage_Datteln_4/LConn3 -- _CN_275138524_380000_CN109504648/RConn3 -- _CN_275138524_380000_CN275138520/LConn3 -- _CN_275138524_380000_CN275138521/LConn3 -- _CN_275138524_380000_CN275138523/LConn3
  G_275138522_/RConn1 -- _CN_275138524_380000_CN275138522/RConn1
  G_275138522_/RConn2 -- _CN_275138524_380000_CN275138522/RConn2
  G_275138522_/RConn3 -- _CN_275138524_380000_CN275138522/RConn3
  G_275138520_/RConn1 -- _CN_275138524_380000_CN275138520/RConn1
  G_275138520_/RConn2 -- _CN_275138524_380000_CN275138520/RConn2
  G_275138520_/RConn3 -- _CN_275138524_380000_CN275138520/RConn3
  G_275138521_/RConn1 -- _CN_275138524_380000_CN275138521/RConn1
  G_275138521_/RConn2 -- _CN_275138524_380000_CN275138521/RConn2
  G_275138521_/RConn3 -- _CN_275138524_380000_CN275138521/RConn3
  G_275138523_/RConn1 -- _CN_275138524_380000_CN275138523/RConn1
  G_275138523_/RConn2 -- _CN_275138524_380000_CN275138523/RConn2
  G_275138523_/RConn3 -- _CN_275138524_380000_CN275138523/RConn3
  T_24258096_380000_Umspannwerk_Hattorf/RConn1 -- L_24258096/LConn1
  T_24258096_380000_Umspannwerk_Hattorf/RConn2 -- L_24258096/LConn2
  T_24258096_380000_Umspannwerk_Hattorf/RConn3 -- L_24258096/LConn3
  T_30017786_220000_Gleidingen_220_kV/RConn1 -- L_30017786/LConn1
  T_30017786_220000_Gleidingen_220_kV/RConn2 -- L_30017786/LConn2
  T_30017786_220000_Gleidingen_220_kV/RConn3 -- L_30017786/LConn3
  T_28227099_220000;110000_Salzgitter_Hallendorf/RConn1 -- L_28227099/LConn1
  T_28227099_220000;110000_Salzgitter_Hallendorf/RConn2 -- L_28227099/LConn2
  T_28227099_220000;110000_Salzgitter_Hallendorf/RConn3 -- L_28227099/LConn3
  T_23899043_380000;110000_Algermissen/RConn1 -- L_23899043/LConn1
  T_23899043_380000;110000_Algermissen/RConn2 -- L_23899043/LConn2
  T_23899043_380000;110000_Algermissen/RConn3 -- L_23899043/LConn3
  T_24413992_380000;110000_UW_Grohnde_380_kV___110_kV/RConn1 -- L_24413992/LConn1
  T_24413992_380000;110000_UW_Grohnde_380_kV___110_kV/RConn2 -- L_24413992/LConn2
  T_24413992_380000;110000_UW_Grohnde_380_kV___110_kV/RConn3 -- L_24413992/LConn3
  T_24272339_380000;110000_Klein_Ilsede/RConn1 -- L_24272339/LConn1
  T_24272339_380000;110000_Klein_Ilsede/RConn2 -- L_24272339/LConn2
  T_24272339_380000;110000_Klein_Ilsede/RConn3 -- L_24272339/LConn3
  T_24272541_220000_Umspannwerk_Braunschweig_Nord/RConn1 -- L_24272541/LConn1
  T_24272541_220000_Umspannwerk_Braunschweig_Nord/RConn2 -- L_24272541/LConn2
  T_24272541_220000_Umspannwerk_Braunschweig_Nord/RConn3 -- L_24272541/LConn3
  T_28343121_380000_Stadorf/RConn1 -- L_28343121/LConn1
  T_28343121_380000_Stadorf/RConn2 -- L_28343121/LConn2
  T_28343121_380000_Stadorf/RConn3 -- L_28343121/LConn3
  T_41334805_220000_Drehstromschaltwerk_Neckarwestheim/RConn1 -- L_41334805/LConn1
  T_41334805_220000_Drehstromschaltwerk_Neckarwestheim/RConn2 -- L_41334805/LConn2
  T_41334805_220000_Drehstromschaltwerk_Neckarwestheim/RConn3 -- L_41334805/LConn3
